simulink model "example"  (R2022a)
settings: Solver=VariableStepAuto  StartTime=0.0  StopTime=10.0  RelTol=1e-3
libraries: kif2 x289
settings Model: Creator=Felhasználó  LastModifiedBy=Felhasználó

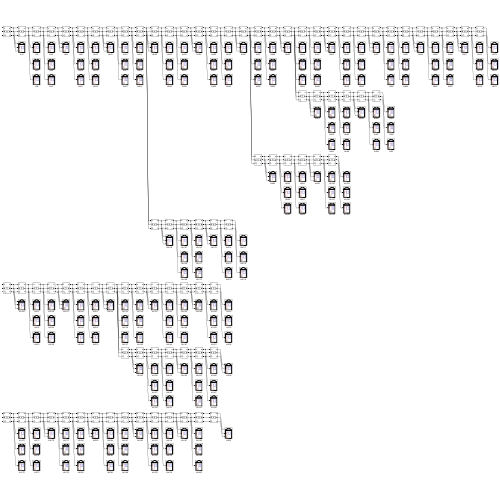
[thumbnail: Simulink's stored preview of the top-level diagram]
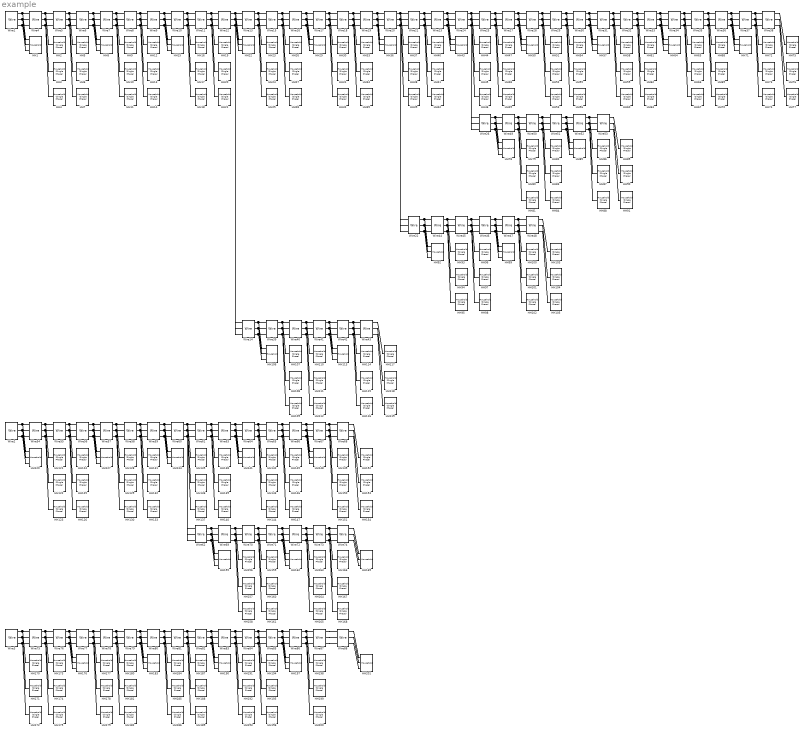
== system example ==
  HH1 : kif2/Household  Ctag=CONS7  Atag=Signal  Itag=Irrad  Ttag=T_Amb  Wtag=Wind  HHtag=PQ_HH1  HHtagv=global  PVtag=PQ_PV1  PVtagv=global  EStag=PQ_ES1  EStagv=global  HPtag=PQ_HP1  HPtagv=global
      link override ES: Cap=36500  SoCin=0.8  Pin=17300  Pout=-17300
      link override HP: P_HP=4800  C=5220  H=284
      link override PV: P_STCm=3100
      settings: SourceProductName=KIF2 Library
  HH10 : kif2/Household (Single Phase)  Ctag=CONS2  Atag=Signal  Itag=Irrad  Ttag=T_Amb  Wtag=Wind  HHtag=PQ_HH10  HHtagv=global  PVtag=PQ_PV10  PVtagv=global  EStag=PQ_ES10  EStagv=global  HPtag=PQ_HP10  HPtagv=global
      link override ES: Cap=13700  SoCin=0.3  Pin=7300  Pout=-7300
      link override HP: P_HP=3000  C=4950  H=141
      link override PV: P_STCm=1200
      settings: SourceProductName=KIF2 Library
  HH100 : kif2/Household (Single Phase)  Ctag=CONS1  Atag=Signal  Itag=Irrad  Ttag=T_Amb  Wtag=Wind  HHtag=PQ_HH100  HHtagv=global  PVtag=PQ_PV100  PVtagv=global  EStag=PQ_ES100  EStagv=global  HPtag=PQ_HP100  HPtagv=global
      link override ES: Cap=9100  SoCin=0.2  Pin=5300  Pout=-5300
      link override HP: P_HP=2400  C=2655  H=140
      link override PV: P_STCm=800
      settings: SourceProductName=KIF2 Library
  HH101 : kif2/Household (Single Phase)  Ctag=CONS2  Atag=Signal  Itag=Irrad  Ttag=T_Amb  Wtag=Wind  HHtag=PQ_HH101  HHtagv=global  PVtag=PQ_PV101  PVtagv=global  EStag=PQ_ES101  EStagv=global  HPtag=PQ_HP101  HPtagv=global
      link override ES: Cap=13700  SoCin=0.3  Pin=7300  Pout=-7300
      link override HP: P_HP=3000  C=4950  H=141
      link override PV: P_STCm=1200
      settings: SourceProductName=KIF2 Library
  HH102 : kif2/Household (Single Phase)  Ctag=CONS3  Atag=Signal  Itag=Irrad  Ttag=T_Amb  Wtag=Wind  HHtag=PQ_HH102  HHtagv=global  PVtag=PQ_PV102  PVtagv=global  EStag=PQ_ES102  EStagv=global  HPtag=PQ_HP102  HPtagv=global
      link override ES: Cap=18300  SoCin=0.4  Pin=9300  Pout=-9300
      link override HP: P_HP=2500  C=2520  H=146
      link override PV: P_STCm=1500
      settings: SourceProductName=KIF2 Library
  HH103 : kif2/Household (Single Phase)  Ctag=CONS4  Atag=Signal  Itag=Irrad  Ttag=T_Amb  Wtag=Wind  HHtag=PQ_HH103  HHtagv=global  PVtag=PQ_PV103  PVtagv=global  EStag=PQ_ES103  EStagv=global  HPtag=PQ_HP103  HPtagv=global
      link override ES: Cap=22800  Pin=11300  Pout=-11300
      link override HP: P_HP=3300  C=4635  H=176
      link override PV: P_STCm=1900
      settings: SourceProductName=KIF2 Library
  HH104 : kif2/Household (Single Phase)  Ctag=CONS5  Atag=Signal  Itag=Irrad  Ttag=T_Amb  Wtag=Wind  HHtag=PQ_HH104  HHtagv=global  PVtag=PQ_PV104  PVtagv=global  EStag=PQ_ES104  EStagv=global  HPtag=PQ_HP104  HPtagv=global
      link override ES: Cap=27400  SoCin=0.6  Pin=13300  Pout=-13300
      link override PV: P_STCm=2300
      settings: SourceProductName=KIF2 Library
  HH105 : kif2/Household (Single Phase)  Ctag=CONS6  Atag=Signal  Itag=Irrad  Ttag=T_Amb  Wtag=Wind  HHtag=PQ_HH105  HHtagv=global  PVtag=PQ_PV105  PVtagv=global  EStag=PQ_ES105  EStagv=global  HPtag=PQ_HP105  HPtagv=global
      link override ES: Cap=32000  SoCin=0.7  Pin=15300  Pout=-15300
      link override HP: P_HP=4200  C=4590  H=241
      settings: SourceProductName=KIF2 Library
  HH106 : kif2/Household  Ctag=CONS7  Atag=Signal  Itag=Irrad  Ttag=T_Amb  Wtag=Wind  HHtag=PQ_HH106  HHtagv=global  PVtag=PQ_PV106  PVtagv=global  EStag=PQ_ES106  EStagv=global  HPtag=PQ_HP106  HPtagv=global
      link override ES: Cap=36500  SoCin=0.8  Pin=17300  Pout=-17300
      link override HP: P_HP=4800  C=5220  H=284
      link override PV: P_STCm=3100
      settings: SourceProductName=KIF2 Library
  HH107 : kif2/Household (Single Phase)  Ctag=CONS1  Atag=Signal  Itag=Irrad  Ttag=T_Amb  Wtag=Wind  HHtag=PQ_HH107  HHtagv=global  PVtag=PQ_PV107  PVtagv=global  EStag=PQ_ES107  EStagv=global  HPtag=PQ_HP107  HPtagv=global
      link override ES: Cap=9100  SoCin=0.2  Pin=5300  Pout=-5300
      link override HP: P_HP=2400  C=2655  H=140
      link override PV: P_STCm=800
      settings: SourceProductName=KIF2 Library
  HH108 : kif2/Household (Single Phase)  Ctag=CONS2  Atag=Signal  Itag=Irrad  Ttag=T_Amb  Wtag=Wind  HHtag=PQ_HH108  HHtagv=global  PVtag=PQ_PV108  PVtagv=global  EStag=PQ_ES108  EStagv=global  HPtag=PQ_HP108  HPtagv=global
      link override ES: Cap=13700  SoCin=0.3  Pin=7300  Pout=-7300
      link override HP: P_HP=3000  C=4950  H=141
      link override PV: P_STCm=1200
      settings: SourceProductName=KIF2 Library
  HH109 : kif2/Household (Single Phase)  Ctag=CONS3  Atag=Signal  Itag=Irrad  Ttag=T_Amb  Wtag=Wind  HHtag=PQ_HH109  HHtagv=global  PVtag=PQ_PV109  PVtagv=global  EStag=PQ_ES109  EStagv=global  HPtag=PQ_HP109  HPtagv=global
      link override ES: Cap=18300  SoCin=0.4  Pin=9300  Pout=-9300
      link override HP: P_HP=2500  C=2520  H=146
      link override PV: P_STCm=1500
      settings: SourceProductName=KIF2 Library
  HH11 : kif2/Household (Single Phase)  Ctag=CONS3  Atag=Signal  Itag=Irrad  Ttag=T_Amb  Wtag=Wind  HHtag=PQ_HH11  HHtagv=global  PVtag=PQ_PV11  PVtagv=global  EStag=PQ_ES11  EStagv=global  HPtag=PQ_HP11  HPtagv=global
      link override ES: Cap=18300  SoCin=0.4  Pin=9300  Pout=-9300
      link override HP: P_HP=2500  C=2520  H=146
      link override PV: P_STCm=1500
      settings: SourceProductName=KIF2 Library
  HH110 : kif2/Household (Single Phase)  Ctag=CONS4  Atag=Signal  Itag=Irrad  Ttag=T_Amb  Wtag=Wind  HHtag=PQ_HH110  HHtagv=global  PVtag=PQ_PV110  PVtagv=global  EStag=PQ_ES110  EStagv=global  HPtag=PQ_HP110  HPtagv=global
      link override ES: Cap=22800  Pin=11300  Pout=-11300
      link override HP: P_HP=3300  C=4635  H=176
      link override PV: P_STCm=1900
      settings: SourceProductName=KIF2 Library
  HH111 : kif2/Household (Single Phase)  Ctag=CONS5  Atag=Signal  Itag=Irrad  Ttag=T_Amb  Wtag=Wind  HHtag=PQ_HH111  HHtagv=global  PVtag=PQ_PV111  PVtagv=global  EStag=PQ_ES111  EStagv=global  HPtag=PQ_HP111  HPtagv=global
      link override ES: Cap=27400  SoCin=0.6  Pin=13300  Pout=-13300
      link override PV: P_STCm=2300
      settings: SourceProductName=KIF2 Library
  HH112 : kif2/Household (Single Phase)  Ctag=CONS6  Atag=Signal  Itag=Irrad  Ttag=T_Amb  Wtag=Wind  HHtag=PQ_HH112  HHtagv=global  PVtag=PQ_PV112  PVtagv=global  EStag=PQ_ES112  EStagv=global  HPtag=PQ_HP112  HPtagv=global
      link override ES: Cap=32000  SoCin=0.7  Pin=15300  Pout=-15300
      link override HP: P_HP=4200  C=4590  H=241
      settings: SourceProductName=KIF2 Library
  HH113 : kif2/Household  Ctag=CONS7  Atag=Signal  Itag=Irrad  Ttag=T_Amb  Wtag=Wind  HHtag=PQ_HH113  HHtagv=global  PVtag=PQ_PV113  PVtagv=global  EStag=PQ_ES113  EStagv=global  HPtag=PQ_HP113  HPtagv=global
      link override ES: Cap=36500  SoCin=0.8  Pin=17300  Pout=-17300
      link override HP: P_HP=4800  C=5220  H=284
      link override PV: P_STCm=3100
      settings: SourceProductName=KIF2 Library
  HH114 : kif2/Household (Single Phase)  Ctag=CONS1  Atag=Signal  Itag=Irrad  Ttag=T_Amb  Wtag=Wind  HHtag=PQ_HH114  HHtagv=global  PVtag=PQ_PV114  PVtagv=global  EStag=PQ_ES114  EStagv=global  HPtag=PQ_HP114  HPtagv=global
      link override ES: Cap=9100  SoCin=0.2  Pin=5300  Pout=-5300
      link override HP: P_HP=2400  C=2655  H=140
      link override PV: P_STCm=800
      settings: SourceProductName=KIF2 Library
  HH115 : kif2/Household (Single Phase)  Ctag=CONS2  Atag=Signal  Itag=Irrad  Ttag=T_Amb  Wtag=Wind  HHtag=PQ_HH115  HHtagv=global  PVtag=PQ_PV115  PVtagv=global  EStag=PQ_ES115  EStagv=global  HPtag=PQ_HP115  HPtagv=global
      link override ES: Cap=13700  SoCin=0.3  Pin=7300  Pout=-7300
      link override HP: P_HP=3000  C=4950  H=141
      link override PV: P_STCm=1200
      settings: SourceProductName=KIF2 Library
  HH116 : kif2/Household (Single Phase)  Ctag=CONS3  Atag=Signal  Itag=Irrad  Ttag=T_Amb  Wtag=Wind  HHtag=PQ_HH116  HHtagv=global  PVtag=PQ_PV116  PVtagv=global  EStag=PQ_ES116  EStagv=global  HPtag=PQ_HP116  HPtagv=global
      link override ES: Cap=18300  SoCin=0.4  Pin=9300  Pout=-9300
      link override HP: P_HP=2500  C=2520  H=146
      link override PV: P_STCm=1500
      settings: SourceProductName=KIF2 Library
  HH117 : kif2/Household (Single Phase)  Ctag=CONS4  Atag=Signal  Itag=Irrad  Ttag=T_Amb  Wtag=Wind  HHtag=PQ_HH117  HHtagv=global  PVtag=PQ_PV117  PVtagv=global  EStag=PQ_ES117  EStagv=global  HPtag=PQ_HP117  HPtagv=global
      link override ES: Cap=22800  Pin=11300  Pout=-11300
      link override HP: P_HP=3300  C=4635  H=176
      link override PV: P_STCm=1900
      settings: SourceProductName=KIF2 Library
  HH118 : kif2/Household (Single Phase)  Ctag=CONS5  Atag=Signal  Itag=Irrad  Ttag=T_Amb  Wtag=Wind  HHtag=PQ_HH118  HHtagv=global  PVtag=PQ_PV118  PVtagv=global  EStag=PQ_ES118  EStagv=global  HPtag=PQ_HP118  HPtagv=global
      link override ES: Cap=27400  SoCin=0.6  Pin=13300  Pout=-13300
      link override PV: P_STCm=2300
      settings: SourceProductName=KIF2 Library
  HH119 : kif2/Household (Single Phase)  Ctag=CONS6  Atag=Signal  Itag=Irrad  Ttag=T_Amb  Wtag=Wind  HHtag=PQ_HH119  HHtagv=global  PVtag=PQ_PV119  PVtagv=global  EStag=PQ_ES119  EStagv=global  HPtag=PQ_HP119  HPtagv=global
      link override ES: Cap=32000  SoCin=0.7  Pin=15300  Pout=-15300
      link override HP: P_HP=4200  C=4590  H=241
      settings: SourceProductName=KIF2 Library
  HH12 : kif2/Household (Single Phase)  Ctag=CONS4  Atag=Signal  Itag=Irrad  Ttag=T_Amb  Wtag=Wind  HHtag=PQ_HH12  HHtagv=global  PVtag=PQ_PV12  PVtagv=global  EStag=PQ_ES12  EStagv=global  HPtag=PQ_HP12  HPtagv=global
      link override ES: Cap=22800  Pin=11300  Pout=-11300
      link override HP: P_HP=3300  C=4635  H=176
      link override PV: P_STCm=1900
      settings: SourceProductName=KIF2 Library
  HH120 : kif2/Household  Ctag=CONS7  Atag=Signal  Itag=Irrad  Ttag=T_Amb  Wtag=Wind  HHtag=PQ_HH120  HHtagv=global  PVtag=PQ_PV120  PVtagv=global  EStag=PQ_ES120  EStagv=global  HPtag=PQ_HP120  HPtagv=global
      link override ES: Cap=36500  SoCin=0.8  Pin=17300  Pout=-17300
      link override HP: P_HP=4800  C=5220  H=284
      link override PV: P_STCm=3100
      settings: SourceProductName=KIF2 Library
  HH121 : kif2/Household (Single Phase)  Ctag=CONS1  Atag=Signal  Itag=Irrad  Ttag=T_Amb  Wtag=Wind  HHtag=PQ_HH121  HHtagv=global  PVtag=PQ_PV121  PVtagv=global  EStag=PQ_ES121  EStagv=global  HPtag=PQ_HP121  HPtagv=global
      link override ES: Cap=9100  SoCin=0.2  Pin=5300  Pout=-5300
      link override HP: P_HP=2400  C=2655  H=140
      link override PV: P_STCm=800
      settings: SourceProductName=KIF2 Library
  HH122 : kif2/Household (Single Phase)  Ctag=CONS2  Atag=Signal  Itag=Irrad  Ttag=T_Amb  Wtag=Wind  HHtag=PQ_HH122  HHtagv=global  PVtag=PQ_PV122  PVtagv=global  EStag=PQ_ES122  EStagv=global  HPtag=PQ_HP122  HPtagv=global
      link override ES: Cap=13700  SoCin=0.3  Pin=7300  Pout=-7300
      link override HP: P_HP=3000  C=4950  H=141
      link override PV: P_STCm=1200
      settings: SourceProductName=KIF2 Library
  HH123 : kif2/Household (Single Phase)  Ctag=CONS3  Atag=Signal  Itag=Irrad  Ttag=T_Amb  Wtag=Wind  HHtag=PQ_HH123  HHtagv=global  PVtag=PQ_PV123  PVtagv=global  EStag=PQ_ES123  EStagv=global  HPtag=PQ_HP123  HPtagv=global
      link override ES: Cap=18300  SoCin=0.4  Pin=9300  Pout=-9300
      link override HP: P_HP=2500  C=2520  H=146
      link override PV: P_STCm=1500
      settings: SourceProductName=KIF2 Library
  HH124 : kif2/Household (Single Phase)  Ctag=CONS4  Atag=Signal  Itag=Irrad  Ttag=T_Amb  Wtag=Wind  HHtag=PQ_HH124  HHtagv=global  PVtag=PQ_PV124  PVtagv=global  EStag=PQ_ES124  EStagv=global  HPtag=PQ_HP124  HPtagv=global
      link override ES: Cap=22800  Pin=11300  Pout=-11300
      link override HP: P_HP=3300  C=4635  H=176
      link override PV: P_STCm=1900
      settings: SourceProductName=KIF2 Library
  HH125 : kif2/Household (Single Phase)  Ctag=CONS5  Atag=Signal  Itag=Irrad  Ttag=T_Amb  Wtag=Wind  HHtag=PQ_HH125  HHtagv=global  PVtag=PQ_PV125  PVtagv=global  EStag=PQ_ES125  EStagv=global  HPtag=PQ_HP125  HPtagv=global
      link override ES: Cap=27400  SoCin=0.6  Pin=13300  Pout=-13300
      link override PV: P_STCm=2300
      settings: SourceProductName=KIF2 Library
  HH126 : kif2/Household (Single Phase)  Ctag=CONS6  Atag=Signal  Itag=Irrad  Ttag=T_Amb  Wtag=Wind  HHtag=PQ_HH126  HHtagv=global  PVtag=PQ_PV126  PVtagv=global  EStag=PQ_ES126  EStagv=global  HPtag=PQ_HP126  HPtagv=global
      link override ES: Cap=32000  SoCin=0.7  Pin=15300  Pout=-15300
      link override HP: P_HP=4200  C=4590  H=241
      settings: SourceProductName=KIF2 Library
  HH127 : kif2/Household  Ctag=CONS7  Atag=Signal  Itag=Irrad  Ttag=T_Amb  Wtag=Wind  HHtag=PQ_HH127  HHtagv=global  PVtag=PQ_PV127  PVtagv=global  EStag=PQ_ES127  EStagv=global  HPtag=PQ_HP127  HPtagv=global
      link override ES: Cap=36500  SoCin=0.8  Pin=17300  Pout=-17300
      link override HP: P_HP=4800  C=5220  H=284
      link override PV: P_STCm=3100
      settings: SourceProductName=KIF2 Library
  HH128 : kif2/Household (Single Phase)  Ctag=CONS1  Atag=Signal  Itag=Irrad  Ttag=T_Amb  Wtag=Wind  HHtag=PQ_HH128  HHtagv=global  PVtag=PQ_PV128  PVtagv=global  EStag=PQ_ES128  EStagv=global  HPtag=PQ_HP128  HPtagv=global
      link override ES: Cap=9100  SoCin=0.2  Pin=5300  Pout=-5300
      link override HP: P_HP=2400  C=2655  H=140
      link override PV: P_STCm=800
      settings: SourceProductName=KIF2 Library
  HH129 : kif2/Household (Single Phase)  Ctag=CONS2  Atag=Signal  Itag=Irrad  Ttag=T_Amb  Wtag=Wind  HHtag=PQ_HH129  HHtagv=global  PVtag=PQ_PV129  PVtagv=global  EStag=PQ_ES129  EStagv=global  HPtag=PQ_HP129  HPtagv=global
      link override ES: Cap=13700  SoCin=0.3  Pin=7300  Pout=-7300
      link override HP: P_HP=3000  C=4950  H=141
      link override PV: P_STCm=1200
      settings: SourceProductName=KIF2 Library
  HH13 : kif2/Household (Single Phase)  Ctag=CONS5  Atag=Signal  Itag=Irrad  Ttag=T_Amb  Wtag=Wind  HHtag=PQ_HH13  HHtagv=global  PVtag=PQ_PV13  PVtagv=global  EStag=PQ_ES13  EStagv=global  HPtag=PQ_HP13  HPtagv=global
      link override ES: Cap=27400  SoCin=0.6  Pin=13300  Pout=-13300
      link override PV: P_STCm=2300
      settings: SourceProductName=KIF2 Library
  HH130 : kif2/Household (Single Phase)  Ctag=CONS3  Atag=Signal  Itag=Irrad  Ttag=T_Amb  Wtag=Wind  HHtag=PQ_HH130  HHtagv=global  PVtag=PQ_PV130  PVtagv=global  EStag=PQ_ES130  EStagv=global  HPtag=PQ_HP130  HPtagv=global
      link override ES: Cap=18300  SoCin=0.4  Pin=9300  Pout=-9300
      link override HP: P_HP=2500  C=2520  H=146
      link override PV: P_STCm=1500
      settings: SourceProductName=KIF2 Library
  HH131 : kif2/Household (Single Phase)  Ctag=CONS4  Atag=Signal  Itag=Irrad  Ttag=T_Amb  Wtag=Wind  HHtag=PQ_HH131  HHtagv=global  PVtag=PQ_PV131  PVtagv=global  EStag=PQ_ES131  EStagv=global  HPtag=PQ_HP131  HPtagv=global
      link override ES: Cap=22800  Pin=11300  Pout=-11300
      link override HP: P_HP=3300  C=4635  H=176
      link override PV: P_STCm=1900
      settings: SourceProductName=KIF2 Library
  HH132 : kif2/Household (Single Phase)  Ctag=CONS5  Atag=Signal  Itag=Irrad  Ttag=T_Amb  Wtag=Wind  HHtag=PQ_HH132  HHtagv=global  PVtag=PQ_PV132  PVtagv=global  EStag=PQ_ES132  EStagv=global  HPtag=PQ_HP132  HPtagv=global
      link override ES: Cap=27400  SoCin=0.6  Pin=13300  Pout=-13300
      link override PV: P_STCm=2300
      settings: SourceProductName=KIF2 Library
  HH133 : kif2/Household (Single Phase)  Ctag=CONS6  Atag=Signal  Itag=Irrad  Ttag=T_Amb  Wtag=Wind  HHtag=PQ_HH133  HHtagv=global  PVtag=PQ_PV133  PVtagv=global  EStag=PQ_ES133  EStagv=global  HPtag=PQ_HP133  HPtagv=global
      link override ES: Cap=32000  SoCin=0.7  Pin=15300  Pout=-15300
      link override HP: P_HP=4200  C=4590  H=241
      settings: SourceProductName=KIF2 Library
  HH134 : kif2/Household  Ctag=CONS7  Atag=Signal  Itag=Irrad  Ttag=T_Amb  Wtag=Wind  HHtag=PQ_HH134  HHtagv=global  PVtag=PQ_PV134  PVtagv=global  EStag=PQ_ES134  EStagv=global  HPtag=PQ_HP134  HPtagv=global
      link override ES: Cap=36500  SoCin=0.8  Pin=17300  Pout=-17300
      link override HP: P_HP=4800  C=5220  H=284
      link override PV: P_STCm=3100
      settings: SourceProductName=KIF2 Library
  HH135 : kif2/Household (Single Phase)  Ctag=CONS1  Atag=Signal  Itag=Irrad  Ttag=T_Amb  Wtag=Wind  HHtag=PQ_HH135  HHtagv=global  PVtag=PQ_PV135  PVtagv=global  EStag=PQ_ES135  EStagv=global  HPtag=PQ_HP135  HPtagv=global
      link override ES: Cap=9100  SoCin=0.2  Pin=5300  Pout=-5300
      link override HP: P_HP=2400  C=2655  H=140
      link override PV: P_STCm=800
      settings: SourceProductName=KIF2 Library
  HH136 : kif2/Household (Single Phase)  Ctag=CONS2  Atag=Signal  Itag=Irrad  Ttag=T_Amb  Wtag=Wind  HHtag=PQ_HH136  HHtagv=global  PVtag=PQ_PV136  PVtagv=global  EStag=PQ_ES136  EStagv=global  HPtag=PQ_HP136  HPtagv=global
      link override ES: Cap=13700  SoCin=0.3  Pin=7300  Pout=-7300
      link override HP: P_HP=3000  C=4950  H=141
      link override PV: P_STCm=1200
      settings: SourceProductName=KIF2 Library
  HH137 : kif2/Household (Single Phase)  Ctag=CONS3  Atag=Signal  Itag=Irrad  Ttag=T_Amb  Wtag=Wind  HHtag=PQ_HH137  HHtagv=global  PVtag=PQ_PV137  PVtagv=global  EStag=PQ_ES137  EStagv=global  HPtag=PQ_HP137  HPtagv=global
      link override ES: Cap=18300  SoCin=0.4  Pin=9300  Pout=-9300
      link override HP: P_HP=2500  C=2520  H=146
      link override PV: P_STCm=1500
      settings: SourceProductName=KIF2 Library
  HH138 : kif2/Household (Single Phase)  Ctag=CONS4  Atag=Signal  Itag=Irrad  Ttag=T_Amb  Wtag=Wind  HHtag=PQ_HH138  HHtagv=global  PVtag=PQ_PV138  PVtagv=global  EStag=PQ_ES138  EStagv=global  HPtag=PQ_HP138  HPtagv=global
      link override ES: Cap=22800  Pin=11300  Pout=-11300
      link override HP: P_HP=3300  C=4635  H=176
      link override PV: P_STCm=1900
      settings: SourceProductName=KIF2 Library
  HH139 : kif2/Household (Single Phase)  Ctag=CONS5  Atag=Signal  Itag=Irrad  Ttag=T_Amb  Wtag=Wind  HHtag=PQ_HH139  HHtagv=global  PVtag=PQ_PV139  PVtagv=global  EStag=PQ_ES139  EStagv=global  HPtag=PQ_HP139  HPtagv=global
      link override ES: Cap=27400  SoCin=0.6  Pin=13300  Pout=-13300
      link override PV: P_STCm=2300
      settings: SourceProductName=KIF2 Library
  HH14 : kif2/Household (Single Phase)  Ctag=CONS6  Atag=Signal  Itag=Irrad  Ttag=T_Amb  Wtag=Wind  HHtag=PQ_HH14  HHtagv=global  PVtag=PQ_PV14  PVtagv=global  EStag=PQ_ES14  EStagv=global  HPtag=PQ_HP14  HPtagv=global
      link override ES: Cap=32000  SoCin=0.7  Pin=15300  Pout=-15300
      link override HP: P_HP=4200  C=4590  H=241
      settings: SourceProductName=KIF2 Library
  HH140 : kif2/Household (Single Phase)  Ctag=CONS6  Atag=Signal  Itag=Irrad  Ttag=T_Amb  Wtag=Wind  HHtag=PQ_HH140  HHtagv=global  PVtag=PQ_PV140  PVtagv=global  EStag=PQ_ES140  EStagv=global  HPtag=PQ_HP140  HPtagv=global
      link override ES: Cap=32000  SoCin=0.7  Pin=15300  Pout=-15300
      link override HP: P_HP=4200  C=4590  H=241
      settings: SourceProductName=KIF2 Library
  HH141 : kif2/Household  Ctag=CONS7  Atag=Signal  Itag=Irrad  Ttag=T_Amb  Wtag=Wind  HHtag=PQ_HH141  HHtagv=global  PVtag=PQ_PV141  PVtagv=global  EStag=PQ_ES141  EStagv=global  HPtag=PQ_HP141  HPtagv=global
      link override ES: Cap=36500  SoCin=0.8  Pin=17300  Pout=-17300
      link override HP: P_HP=4800  C=5220  H=284
      link override PV: P_STCm=3100
      settings: SourceProductName=KIF2 Library
  HH142 : kif2/Household (Single Phase)  Ctag=CONS1  Atag=Signal  Itag=Irrad  Ttag=T_Amb  Wtag=Wind  HHtag=PQ_HH142  HHtagv=global  PVtag=PQ_PV142  PVtagv=global  EStag=PQ_ES142  EStagv=global  HPtag=PQ_HP142  HPtagv=global
      link override ES: Cap=9100  SoCin=0.2  Pin=5300  Pout=-5300
      link override HP: P_HP=2400  C=2655  H=140
      link override PV: P_STCm=800
      settings: SourceProductName=KIF2 Library
  HH143 : kif2/Household (Single Phase)  Ctag=CONS2  Atag=Signal  Itag=Irrad  Ttag=T_Amb  Wtag=Wind  HHtag=PQ_HH143  HHtagv=global  PVtag=PQ_PV143  PVtagv=global  EStag=PQ_ES143  EStagv=global  HPtag=PQ_HP143  HPtagv=global
      link override ES: Cap=13700  SoCin=0.3  Pin=7300  Pout=-7300
      link override HP: P_HP=3000  C=4950  H=141
      link override PV: P_STCm=1200
      settings: SourceProductName=KIF2 Library
  HH144 : kif2/Household (Single Phase)  Ctag=CONS3  Atag=Signal  Itag=Irrad  Ttag=T_Amb  Wtag=Wind  HHtag=PQ_HH144  HHtagv=global  PVtag=PQ_PV144  PVtagv=global  EStag=PQ_ES144  EStagv=global  HPtag=PQ_HP144  HPtagv=global
      link override ES: Cap=18300  SoCin=0.4  Pin=9300  Pout=-9300
      link override HP: P_HP=2500  C=2520  H=146
      link override PV: P_STCm=1500
      settings: SourceProductName=KIF2 Library
  HH145 : kif2/Household (Single Phase)  Ctag=CONS4  Atag=Signal  Itag=Irrad  Ttag=T_Amb  Wtag=Wind  HHtag=PQ_HH145  HHtagv=global  PVtag=PQ_PV145  PVtagv=global  EStag=PQ_ES145  EStagv=global  HPtag=PQ_HP145  HPtagv=global
      link override ES: Cap=22800  Pin=11300  Pout=-11300
      link override HP: P_HP=3300  C=4635  H=176
      link override PV: P_STCm=1900
      settings: SourceProductName=KIF2 Library
  HH146 : kif2/Household (Single Phase)  Ctag=CONS5  Atag=Signal  Itag=Irrad  Ttag=T_Amb  Wtag=Wind  HHtag=PQ_HH146  HHtagv=global  PVtag=PQ_PV146  PVtagv=global  EStag=PQ_ES146  EStagv=global  HPtag=PQ_HP146  HPtagv=global
      link override ES: Cap=27400  SoCin=0.6  Pin=13300  Pout=-13300
      link override PV: P_STCm=2300
      settings: SourceProductName=KIF2 Library
  HH147 : kif2/Household (Single Phase)  Ctag=CONS6  Atag=Signal  Itag=Irrad  Ttag=T_Amb  Wtag=Wind  HHtag=PQ_HH147  HHtagv=global  PVtag=PQ_PV147  PVtagv=global  EStag=PQ_ES147  EStagv=global  HPtag=PQ_HP147  HPtagv=global
      link override ES: Cap=32000  SoCin=0.7  Pin=15300  Pout=-15300
      link override HP: P_HP=4200  C=4590  H=241
      settings: SourceProductName=KIF2 Library
  HH148 : kif2/Household  Ctag=CONS7  Atag=Signal  Itag=Irrad  Ttag=T_Amb  Wtag=Wind  HHtag=PQ_HH148  HHtagv=global  PVtag=PQ_PV148  PVtagv=global  EStag=PQ_ES148  EStagv=global  HPtag=PQ_HP148  HPtagv=global
      link override ES: Cap=36500  SoCin=0.8  Pin=17300  Pout=-17300
      link override HP: P_HP=4800  C=5220  H=284
      link override PV: P_STCm=3100
      settings: SourceProductName=KIF2 Library
  HH149 : kif2/Household (Single Phase)  Ctag=CONS1  Atag=Signal  Itag=Irrad  Ttag=T_Amb  Wtag=Wind  HHtag=PQ_HH149  HHtagv=global  PVtag=PQ_PV149  PVtagv=global  EStag=PQ_ES149  EStagv=global  HPtag=PQ_HP149  HPtagv=global
      link override ES: Cap=9100  SoCin=0.2  Pin=5300  Pout=-5300
      link override HP: P_HP=2400  C=2655  H=140
      link override PV: P_STCm=800
      settings: SourceProductName=KIF2 Library
  HH15 : kif2/Household  Ctag=CONS7  Atag=Signal  Itag=Irrad  Ttag=T_Amb  Wtag=Wind  HHtag=PQ_HH15  HHtagv=global  PVtag=PQ_PV15  PVtagv=global  EStag=PQ_ES15  EStagv=global  HPtag=PQ_HP15  HPtagv=global
      link override ES: Cap=36500  SoCin=0.8  Pin=17300  Pout=-17300
      link override HP: P_HP=4800  C=5220  H=284
      link override PV: P_STCm=3100
      settings: SourceProductName=KIF2 Library
  HH150 : kif2/Household (Single Phase)  Ctag=CONS2  Atag=Signal  Itag=Irrad  Ttag=T_Amb  Wtag=Wind  HHtag=PQ_HH150  HHtagv=global  PVtag=PQ_PV150  PVtagv=global  EStag=PQ_ES150  EStagv=global  HPtag=PQ_HP150  HPtagv=global
      link override ES: Cap=13700  SoCin=0.3  Pin=7300  Pout=-7300
      link override HP: P_HP=3000  C=4950  H=141
      link override PV: P_STCm=1200
      settings: SourceProductName=KIF2 Library
  HH151 : kif2/Household (Single Phase)  Ctag=CONS3  Atag=Signal  Itag=Irrad  Ttag=T_Amb  Wtag=Wind  HHtag=PQ_HH151  HHtagv=global  PVtag=PQ_PV151  PVtagv=global  EStag=PQ_ES151  EStagv=global  HPtag=PQ_HP151  HPtagv=global
      link override ES: Cap=18300  SoCin=0.4  Pin=9300  Pout=-9300
      link override HP: P_HP=2500  C=2520  H=146
      link override PV: P_STCm=1500
      settings: SourceProductName=KIF2 Library
  HH152 : kif2/Household (Single Phase)  Ctag=CONS4  Atag=Signal  Itag=Irrad  Ttag=T_Amb  Wtag=Wind  HHtag=PQ_HH152  HHtagv=global  PVtag=PQ_PV152  PVtagv=global  EStag=PQ_ES152  EStagv=global  HPtag=PQ_HP152  HPtagv=global
      link override ES: Cap=22800  Pin=11300  Pout=-11300
      link override HP: P_HP=3300  C=4635  H=176
      link override PV: P_STCm=1900
      settings: SourceProductName=KIF2 Library
  HH153 : kif2/Household (Single Phase)  Ctag=CONS5  Atag=Signal  Itag=Irrad  Ttag=T_Amb  Wtag=Wind  HHtag=PQ_HH153  HHtagv=global  PVtag=PQ_PV153  PVtagv=global  EStag=PQ_ES153  EStagv=global  HPtag=PQ_HP153  HPtagv=global
      link override ES: Cap=27400  SoCin=0.6  Pin=13300  Pout=-13300
      link override PV: P_STCm=2300
      settings: SourceProductName=KIF2 Library
  HH154 : kif2/Household (Single Phase)  Ctag=CONS6  Atag=Signal  Itag=Irrad  Ttag=T_Amb  Wtag=Wind  HHtag=PQ_HH154  HHtagv=global  PVtag=PQ_PV154  PVtagv=global  EStag=PQ_ES154  EStagv=global  HPtag=PQ_HP154  HPtagv=global
      link override ES: Cap=32000  SoCin=0.7  Pin=15300  Pout=-15300
      link override HP: P_HP=4200  C=4590  H=241
      settings: SourceProductName=KIF2 Library
  HH155 : kif2/Household  Ctag=CONS7  Atag=Signal  Itag=Irrad  Ttag=T_Amb  Wtag=Wind  HHtag=PQ_HH155  HHtagv=global  PVtag=PQ_PV155  PVtagv=global  EStag=PQ_ES155  EStagv=global  HPtag=PQ_HP155  HPtagv=global
      link override ES: Cap=36500  SoCin=0.8  Pin=17300  Pout=-17300
      link override HP: P_HP=4800  C=5220  H=284
      link override PV: P_STCm=3100
      settings: SourceProductName=KIF2 Library
  HH156 : kif2/Household (Single Phase)  Ctag=CONS1  Atag=Signal  Itag=Irrad  Ttag=T_Amb  Wtag=Wind  HHtag=PQ_HH156  HHtagv=global  PVtag=PQ_PV156  PVtagv=global  EStag=PQ_ES156  EStagv=global  HPtag=PQ_HP156  HPtagv=global
      link override ES: Cap=9100  SoCin=0.2  Pin=5300  Pout=-5300
      link override HP: P_HP=2400  C=2655  H=140
      link override PV: P_STCm=800
      settings: SourceProductName=KIF2 Library
  HH157 : kif2/Household (Single Phase)  Ctag=CONS2  Atag=Signal  Itag=Irrad  Ttag=T_Amb  Wtag=Wind  HHtag=PQ_HH157  HHtagv=global  PVtag=PQ_PV157  PVtagv=global  EStag=PQ_ES157  EStagv=global  HPtag=PQ_HP157  HPtagv=global
      link override ES: Cap=13700  SoCin=0.3  Pin=7300  Pout=-7300
      link override HP: P_HP=3000  C=4950  H=141
      link override PV: P_STCm=1200
      settings: SourceProductName=KIF2 Library
  HH158 : kif2/Household (Single Phase)  Ctag=CONS3  Atag=Signal  Itag=Irrad  Ttag=T_Amb  Wtag=Wind  HHtag=PQ_HH158  HHtagv=global  PVtag=PQ_PV158  PVtagv=global  EStag=PQ_ES158  EStagv=global  HPtag=PQ_HP158  HPtagv=global
      link override ES: Cap=18300  SoCin=0.4  Pin=9300  Pout=-9300
      link override HP: P_HP=2500  C=2520  H=146
      link override PV: P_STCm=1500
      settings: SourceProductName=KIF2 Library
  HH159 : kif2/Household (Single Phase)  Ctag=CONS4  Atag=Signal  Itag=Irrad  Ttag=T_Amb  Wtag=Wind  HHtag=PQ_HH159  HHtagv=global  PVtag=PQ_PV159  PVtagv=global  EStag=PQ_ES159  EStagv=global  HPtag=PQ_HP159  HPtagv=global
      link override ES: Cap=22800  Pin=11300  Pout=-11300
      link override HP: P_HP=3300  C=4635  H=176
      link override PV: P_STCm=1900
      settings: SourceProductName=KIF2 Library
  HH16 : kif2/Household (Single Phase)  Ctag=CONS1  Atag=Signal  Itag=Irrad  Ttag=T_Amb  Wtag=Wind  HHtag=PQ_HH16  HHtagv=global  PVtag=PQ_PV16  PVtagv=global  EStag=PQ_ES16  EStagv=global  HPtag=PQ_HP16  HPtagv=global
      link override ES: Cap=9100  SoCin=0.2  Pin=5300  Pout=-5300
      link override HP: P_HP=2400  C=2655  H=140
      link override PV: P_STCm=800
      settings: SourceProductName=KIF2 Library
  HH160 : kif2/Household (Single Phase)  Ctag=CONS5  Atag=Signal  Itag=Irrad  Ttag=T_Amb  Wtag=Wind  HHtag=PQ_HH160  HHtagv=global  PVtag=PQ_PV160  PVtagv=global  EStag=PQ_ES160  EStagv=global  HPtag=PQ_HP160  HPtagv=global
      link override ES: Cap=27400  SoCin=0.6  Pin=13300  Pout=-13300
      link override PV: P_STCm=2300
      settings: SourceProductName=KIF2 Library
  HH161 : kif2/Household (Single Phase)  Ctag=CONS6  Atag=Signal  Itag=Irrad  Ttag=T_Amb  Wtag=Wind  HHtag=PQ_HH161  HHtagv=global  PVtag=PQ_PV161  PVtagv=global  EStag=PQ_ES161  EStagv=global  HPtag=PQ_HP161  HPtagv=global
      link override ES: Cap=32000  SoCin=0.7  Pin=15300  Pout=-15300
      link override HP: P_HP=4200  C=4590  H=241
      settings: SourceProductName=KIF2 Library
  HH162 : kif2/Household  Ctag=CONS7  Atag=Signal  Itag=Irrad  Ttag=T_Amb  Wtag=Wind  HHtag=PQ_HH162  HHtagv=global  PVtag=PQ_PV162  PVtagv=global  EStag=PQ_ES162  EStagv=global  HPtag=PQ_HP162  HPtagv=global
      link override ES: Cap=36500  SoCin=0.8  Pin=17300  Pout=-17300
      link override HP: P_HP=4800  C=5220  H=284
      link override PV: P_STCm=3100
      settings: SourceProductName=KIF2 Library
  HH163 : kif2/Household (Single Phase)  Ctag=CONS1  Atag=Signal  Itag=Irrad  Ttag=T_Amb  Wtag=Wind  HHtag=PQ_HH163  HHtagv=global  PVtag=PQ_PV163  PVtagv=global  EStag=PQ_ES163  EStagv=global  HPtag=PQ_HP163  HPtagv=global
      link override ES: Cap=9100  SoCin=0.2  Pin=5300  Pout=-5300
      link override HP: P_HP=2400  C=2655  H=140
      link override PV: P_STCm=800
      settings: SourceProductName=KIF2 Library
  HH164 : kif2/Household (Single Phase)  Ctag=CONS2  Atag=Signal  Itag=Irrad  Ttag=T_Amb  Wtag=Wind  HHtag=PQ_HH164  HHtagv=global  PVtag=PQ_PV164  PVtagv=global  EStag=PQ_ES164  EStagv=global  HPtag=PQ_HP164  HPtagv=global
      link override ES: Cap=13700  SoCin=0.3  Pin=7300  Pout=-7300
      link override HP: P_HP=3000  C=4950  H=141
      link override PV: P_STCm=1200
      settings: SourceProductName=KIF2 Library
  HH165 : kif2/Household (Single Phase)  Ctag=CONS3  Atag=Signal  Itag=Irrad  Ttag=T_Amb  Wtag=Wind  HHtag=PQ_HH165  HHtagv=global  PVtag=PQ_PV165  PVtagv=global  EStag=PQ_ES165  EStagv=global  HPtag=PQ_HP165  HPtagv=global
      link override ES: Cap=18300  SoCin=0.4  Pin=9300  Pout=-9300
      link override HP: P_HP=2500  C=2520  H=146
      link override PV: P_STCm=1500
      settings: SourceProductName=KIF2 Library
  HH166 : kif2/Household (Single Phase)  Ctag=CONS4  Atag=Signal  Itag=Irrad  Ttag=T_Amb  Wtag=Wind  HHtag=PQ_HH166  HHtagv=global  PVtag=PQ_PV166  PVtagv=global  EStag=PQ_ES166  EStagv=global  HPtag=PQ_HP166  HPtagv=global
      link override ES: Cap=22800  Pin=11300  Pout=-11300
      link override HP: P_HP=3300  C=4635  H=176
      link override PV: P_STCm=1900
      settings: SourceProductName=KIF2 Library
  HH167 : kif2/Household (Single Phase)  Ctag=CONS5  Atag=Signal  Itag=Irrad  Ttag=T_Amb  Wtag=Wind  HHtag=PQ_HH167  HHtagv=global  PVtag=PQ_PV167  PVtagv=global  EStag=PQ_ES167  EStagv=global  HPtag=PQ_HP167  HPtagv=global
      link override ES: Cap=27400  SoCin=0.6  Pin=13300  Pout=-13300
      link override PV: P_STCm=2300
      settings: SourceProductName=KIF2 Library
  HH168 : kif2/Household (Single Phase)  Ctag=CONS6  Atag=Signal  Itag=Irrad  Ttag=T_Amb  Wtag=Wind  HHtag=PQ_HH168  HHtagv=global  PVtag=PQ_PV168  PVtagv=global  EStag=PQ_ES168  EStagv=global  HPtag=PQ_HP168  HPtagv=global
      link override ES: Cap=32000  SoCin=0.7  Pin=15300  Pout=-15300
      link override HP: P_HP=4200  C=4590  H=241
      settings: SourceProductName=KIF2 Library
  HH169 : kif2/Household  Ctag=CONS7  Atag=Signal  Itag=Irrad  Ttag=T_Amb  Wtag=Wind  HHtag=PQ_HH169  HHtagv=global  PVtag=PQ_PV169  PVtagv=global  EStag=PQ_ES169  EStagv=global  HPtag=PQ_HP169  HPtagv=global
      link override ES: Cap=36500  SoCin=0.8  Pin=17300  Pout=-17300
      link override HP: P_HP=4800  C=5220  H=284
      link override PV: P_STCm=3100
      settings: SourceProductName=KIF2 Library
  HH17 : kif2/Household (Single Phase)  Ctag=CONS2  Atag=Signal  Itag=Irrad  Ttag=T_Amb  Wtag=Wind  HHtag=PQ_HH17  HHtagv=global  PVtag=PQ_PV17  PVtagv=global  EStag=PQ_ES17  EStagv=global  HPtag=PQ_HP17  HPtagv=global
      link override ES: Cap=13700  SoCin=0.3  Pin=7300  Pout=-7300
      link override HP: P_HP=3000  C=4950  H=141
      link override PV: P_STCm=1200
      settings: SourceProductName=KIF2 Library
  HH170 : kif2/Household (Single Phase)  Ctag=CONS1  Atag=Signal  Itag=Irrad  Ttag=T_Amb  Wtag=Wind  HHtag=PQ_HH170  HHtagv=global  PVtag=PQ_PV170  PVtagv=global  EStag=PQ_ES170  EStagv=global  HPtag=PQ_HP170  HPtagv=global
      link override ES: Cap=9100  SoCin=0.2  Pin=5300  Pout=-5300
      link override HP: P_HP=2400  C=2655  H=140
      link override PV: P_STCm=800
      settings: SourceProductName=KIF2 Library
  HH171 : kif2/Household (Single Phase)  Ctag=CONS2  Atag=Signal  Itag=Irrad  Ttag=T_Amb  Wtag=Wind  HHtag=PQ_HH171  HHtagv=global  PVtag=PQ_PV171  PVtagv=global  EStag=PQ_ES171  EStagv=global  HPtag=PQ_HP171  HPtagv=global
      link override ES: Cap=13700  SoCin=0.3  Pin=7300  Pout=-7300
      link override HP: P_HP=3000  C=4950  H=141
      link override PV: P_STCm=1200
      settings: SourceProductName=KIF2 Library
  HH172 : kif2/Household (Single Phase)  Ctag=CONS3  Atag=Signal  Itag=Irrad  Ttag=T_Amb  Wtag=Wind  HHtag=PQ_HH172  HHtagv=global  PVtag=PQ_PV172  PVtagv=global  EStag=PQ_ES172  EStagv=global  HPtag=PQ_HP172  HPtagv=global
      link override ES: Cap=18300  SoCin=0.4  Pin=9300  Pout=-9300
      link override HP: P_HP=2500  C=2520  H=146
      link override PV: P_STCm=1500
      settings: SourceProductName=KIF2 Library
  HH173 : kif2/Household (Single Phase)  Ctag=CONS4  Atag=Signal  Itag=Irrad  Ttag=T_Amb  Wtag=Wind  HHtag=PQ_HH173  HHtagv=global  PVtag=PQ_PV173  PVtagv=global  EStag=PQ_ES173  EStagv=global  HPtag=PQ_HP173  HPtagv=global
      link override ES: Cap=22800  Pin=11300  Pout=-11300
      link override HP: P_HP=3300  C=4635  H=176
      link override PV: P_STCm=1900
      settings: SourceProductName=KIF2 Library
  HH174 : kif2/Household (Single Phase)  Ctag=CONS5  Atag=Signal  Itag=Irrad  Ttag=T_Amb  Wtag=Wind  HHtag=PQ_HH174  HHtagv=global  PVtag=PQ_PV174  PVtagv=global  EStag=PQ_ES174  EStagv=global  HPtag=PQ_HP174  HPtagv=global
      link override ES: Cap=27400  SoCin=0.6  Pin=13300  Pout=-13300
      link override PV: P_STCm=2300
      settings: SourceProductName=KIF2 Library
  HH175 : kif2/Household (Single Phase)  Ctag=CONS6  Atag=Signal  Itag=Irrad  Ttag=T_Amb  Wtag=Wind  HHtag=PQ_HH175  HHtagv=global  PVtag=PQ_PV175  PVtagv=global  EStag=PQ_ES175  EStagv=global  HPtag=PQ_HP175  HPtagv=global
      link override ES: Cap=32000  SoCin=0.7  Pin=15300  Pout=-15300
      link override HP: P_HP=4200  C=4590  H=241
      settings: SourceProductName=KIF2 Library
  HH176 : kif2/Household  Ctag=CONS7  Atag=Signal  Itag=Irrad  Ttag=T_Amb  Wtag=Wind  HHtag=PQ_HH176  HHtagv=global  PVtag=PQ_PV176  PVtagv=global  EStag=PQ_ES176  EStagv=global  HPtag=PQ_HP176  HPtagv=global
      link override ES: Cap=36500  SoCin=0.8  Pin=17300  Pout=-17300
      link override HP: P_HP=4800  C=5220  H=284
      link override PV: P_STCm=3100
      settings: SourceProductName=KIF2 Library
  HH177 : kif2/Household (Single Phase)  Ctag=CONS1  Atag=Signal  Itag=Irrad  Ttag=T_Amb  Wtag=Wind  HHtag=PQ_HH177  HHtagv=global  PVtag=PQ_PV177  PVtagv=global  EStag=PQ_ES177  EStagv=global  HPtag=PQ_HP177  HPtagv=global
      link override ES: Cap=9100  SoCin=0.2  Pin=5300  Pout=-5300
      link override HP: P_HP=2400  C=2655  H=140
      link override PV: P_STCm=800
      settings: SourceProductName=KIF2 Library
  HH178 : kif2/Household (Single Phase)  Ctag=CONS2  Atag=Signal  Itag=Irrad  Ttag=T_Amb  Wtag=Wind  HHtag=PQ_HH178  HHtagv=global  PVtag=PQ_PV178  PVtagv=global  EStag=PQ_ES178  EStagv=global  HPtag=PQ_HP178  HPtagv=global
      link override ES: Cap=13700  SoCin=0.3  Pin=7300  Pout=-7300
      link override HP: P_HP=3000  C=4950  H=141
      link override PV: P_STCm=1200
      settings: SourceProductName=KIF2 Library
  HH179 : kif2/Household (Single Phase)  Ctag=CONS3  Atag=Signal  Itag=Irrad  Ttag=T_Amb  Wtag=Wind  HHtag=PQ_HH179  HHtagv=global  PVtag=PQ_PV179  PVtagv=global  EStag=PQ_ES179  EStagv=global  HPtag=PQ_HP179  HPtagv=global
      link override ES: Cap=18300  SoCin=0.4  Pin=9300  Pout=-9300
      link override HP: P_HP=2500  C=2520  H=146
      link override PV: P_STCm=1500
      settings: SourceProductName=KIF2 Library
  HH18 : kif2/Household (Single Phase)  Ctag=CONS3  Atag=Signal  Itag=Irrad  Ttag=T_Amb  Wtag=Wind  HHtag=PQ_HH18  HHtagv=global  PVtag=PQ_PV18  PVtagv=global  EStag=PQ_ES18  EStagv=global  HPtag=PQ_HP18  HPtagv=global
      link override ES: Cap=18300  SoCin=0.4  Pin=9300  Pout=-9300
      link override HP: P_HP=2500  C=2520  H=146
      link override PV: P_STCm=1500
      settings: SourceProductName=KIF2 Library
  HH180 : kif2/Household (Single Phase)  Ctag=CONS4  Atag=Signal  Itag=Irrad  Ttag=T_Amb  Wtag=Wind  HHtag=PQ_HH180  HHtagv=global  PVtag=PQ_PV180  PVtagv=global  EStag=PQ_ES180  EStagv=global  HPtag=PQ_HP180  HPtagv=global
      link override ES: Cap=22800  Pin=11300  Pout=-11300
      link override HP: P_HP=3300  C=4635  H=176
      link override PV: P_STCm=1900
      settings: SourceProductName=KIF2 Library
  HH181 : kif2/Household (Single Phase)  Ctag=CONS5  Atag=Signal  Itag=Irrad  Ttag=T_Amb  Wtag=Wind  HHtag=PQ_HH181  HHtagv=global  PVtag=PQ_PV181  PVtagv=global  EStag=PQ_ES181  EStagv=global  HPtag=PQ_HP181  HPtagv=global
      link override ES: Cap=27400  SoCin=0.6  Pin=13300  Pout=-13300
      link override PV: P_STCm=2300
      settings: SourceProductName=KIF2 Library
  HH182 : kif2/Household (Single Phase)  Ctag=CONS6  Atag=Signal  Itag=Irrad  Ttag=T_Amb  Wtag=Wind  HHtag=PQ_HH182  HHtagv=global  PVtag=PQ_PV182  PVtagv=global  EStag=PQ_ES182  EStagv=global  HPtag=PQ_HP182  HPtagv=global
      link override ES: Cap=32000  SoCin=0.7  Pin=15300  Pout=-15300
      link override HP: P_HP=4200  C=4590  H=241
      settings: SourceProductName=KIF2 Library
  HH183 : kif2/Household  Ctag=CONS7  Atag=Signal  Itag=Irrad  Ttag=T_Amb  Wtag=Wind  HHtag=PQ_HH183  HHtagv=global  PVtag=PQ_PV183  PVtagv=global  EStag=PQ_ES183  EStagv=global  HPtag=PQ_HP183  HPtagv=global
      link override ES: Cap=36500  SoCin=0.8  Pin=17300  Pout=-17300
      link override HP: P_HP=4800  C=5220  H=284
      link override PV: P_STCm=3100
      settings: SourceProductName=KIF2 Library
  HH184 : kif2/Household (Single Phase)  Ctag=CONS1  Atag=Signal  Itag=Irrad  Ttag=T_Amb  Wtag=Wind  HHtag=PQ_HH184  HHtagv=global  PVtag=PQ_PV184  PVtagv=global  EStag=PQ_ES184  EStagv=global  HPtag=PQ_HP184  HPtagv=global
      link override ES: Cap=9100  SoCin=0.2  Pin=5300  Pout=-5300
      link override HP: P_HP=2400  C=2655  H=140
      link override PV: P_STCm=800
      settings: SourceProductName=KIF2 Library
  HH185 : kif2/Household (Single Phase)  Ctag=CONS2  Atag=Signal  Itag=Irrad  Ttag=T_Amb  Wtag=Wind  HHtag=PQ_HH185  HHtagv=global  PVtag=PQ_PV185  PVtagv=global  EStag=PQ_ES185  EStagv=global  HPtag=PQ_HP185  HPtagv=global
      link override ES: Cap=13700  SoCin=0.3  Pin=7300  Pout=-7300
      link override HP: P_HP=3000  C=4950  H=141
      link override PV: P_STCm=1200
      settings: SourceProductName=KIF2 Library
  HH186 : kif2/Household (Single Phase)  Ctag=CONS3  Atag=Signal  Itag=Irrad  Ttag=T_Amb  Wtag=Wind  HHtag=PQ_HH186  HHtagv=global  PVtag=PQ_PV186  PVtagv=global  EStag=PQ_ES186  EStagv=global  HPtag=PQ_HP186  HPtagv=global
      link override ES: Cap=18300  SoCin=0.4  Pin=9300  Pout=-9300
      link override HP: P_HP=2500  C=2520  H=146
      link override PV: P_STCm=1500
      settings: SourceProductName=KIF2 Library
  HH187 : kif2/Household (Single Phase)  Ctag=CONS4  Atag=Signal  Itag=Irrad  Ttag=T_Amb  Wtag=Wind  HHtag=PQ_HH187  HHtagv=global  PVtag=PQ_PV187  PVtagv=global  EStag=PQ_ES187  EStagv=global  HPtag=PQ_HP187  HPtagv=global
      link override ES: Cap=22800  Pin=11300  Pout=-11300
      link override HP: P_HP=3300  C=4635  H=176
      link override PV: P_STCm=1900
      settings: SourceProductName=KIF2 Library
  HH188 : kif2/Household (Single Phase)  Ctag=CONS5  Atag=Signal  Itag=Irrad  Ttag=T_Amb  Wtag=Wind  HHtag=PQ_HH188  HHtagv=global  PVtag=PQ_PV188  PVtagv=global  EStag=PQ_ES188  EStagv=global  HPtag=PQ_HP188  HPtagv=global
      link override ES: Cap=27400  SoCin=0.6  Pin=13300  Pout=-13300
      link override PV: P_STCm=2300
      settings: SourceProductName=KIF2 Library
  HH189 : kif2/Household (Single Phase)  Ctag=CONS6  Atag=Signal  Itag=Irrad  Ttag=T_Amb  Wtag=Wind  HHtag=PQ_HH189  HHtagv=global  PVtag=PQ_PV189  PVtagv=global  EStag=PQ_ES189  EStagv=global  HPtag=PQ_HP189  HPtagv=global
      link override ES: Cap=32000  SoCin=0.7  Pin=15300  Pout=-15300
      link override HP: P_HP=4200  C=4590  H=241
      settings: SourceProductName=KIF2 Library
  HH19 : kif2/Household (Single Phase)  Ctag=CONS4  Atag=Signal  Itag=Irrad  Ttag=T_Amb  Wtag=Wind  HHtag=PQ_HH19  HHtagv=global  PVtag=PQ_PV19  PVtagv=global  EStag=PQ_ES19  EStagv=global  HPtag=PQ_HP19  HPtagv=global
      link override ES: Cap=22800  Pin=11300  Pout=-11300
      link override HP: P_HP=3300  C=4635  H=176
      link override PV: P_STCm=1900
      settings: SourceProductName=KIF2 Library
  HH190 : kif2/Household  Ctag=CONS7  Atag=Signal  Itag=Irrad  Ttag=T_Amb  Wtag=Wind  HHtag=PQ_HH190  HHtagv=global  PVtag=PQ_PV190  PVtagv=global  EStag=PQ_ES190  EStagv=global  HPtag=PQ_HP190  HPtagv=global
      link override ES: Cap=36500  SoCin=0.8  Pin=17300  Pout=-17300
      link override HP: P_HP=4800  C=5220  H=284
      link override PV: P_STCm=3100
      settings: SourceProductName=KIF2 Library
  HH191 : kif2/Household (Single Phase)  Ctag=CONS1  Atag=Signal  Itag=Irrad  Ttag=T_Amb  Wtag=Wind  HHtag=PQ_HH191  HHtagv=global  PVtag=PQ_PV191  PVtagv=global  EStag=PQ_ES191  EStagv=global  HPtag=PQ_HP191  HPtagv=global
      link override ES: Cap=9100  SoCin=0.2  Pin=5300  Pout=-5300
      link override HP: P_HP=2400  C=2655  H=140
      link override PV: P_STCm=800
      settings: SourceProductName=KIF2 Library
  HH192 : kif2/Household (Single Phase)  Ctag=CONS2  Atag=Signal  Itag=Irrad  Ttag=T_Amb  Wtag=Wind  HHtag=PQ_HH192  HHtagv=global  PVtag=PQ_PV192  PVtagv=global  EStag=PQ_ES192  EStagv=global  HPtag=PQ_HP192  HPtagv=global
      link override ES: Cap=13700  SoCin=0.3  Pin=7300  Pout=-7300
      link override HP: P_HP=3000  C=4950  H=141
      link override PV: P_STCm=1200
      settings: SourceProductName=KIF2 Library
  HH193 : kif2/Household (Single Phase)  Ctag=CONS3  Atag=Signal  Itag=Irrad  Ttag=T_Amb  Wtag=Wind  HHtag=PQ_HH193  HHtagv=global  PVtag=PQ_PV193  PVtagv=global  EStag=PQ_ES193  EStagv=global  HPtag=PQ_HP193  HPtagv=global
      link override ES: Cap=18300  SoCin=0.4  Pin=9300  Pout=-9300
      link override HP: P_HP=2500  C=2520  H=146
      link override PV: P_STCm=1500
      settings: SourceProductName=KIF2 Library
  HH194 : kif2/Household (Single Phase)  Ctag=CONS4  Atag=Signal  Itag=Irrad  Ttag=T_Amb  Wtag=Wind  HHtag=PQ_HH194  HHtagv=global  PVtag=PQ_PV194  PVtagv=global  EStag=PQ_ES194  EStagv=global  HPtag=PQ_HP194  HPtagv=global
      link override ES: Cap=22800  Pin=11300  Pout=-11300
      link override HP: P_HP=3300  C=4635  H=176
      link override PV: P_STCm=1900
      settings: SourceProductName=KIF2 Library
  HH195 : kif2/Household (Single Phase)  Ctag=CONS5  Atag=Signal  Itag=Irrad  Ttag=T_Amb  Wtag=Wind  HHtag=PQ_HH195  HHtagv=global  PVtag=PQ_PV195  PVtagv=global  EStag=PQ_ES195  EStagv=global  HPtag=PQ_HP195  HPtagv=global
      link override ES: Cap=27400  SoCin=0.6  Pin=13300  Pout=-13300
      link override PV: P_STCm=2300
      settings: SourceProductName=KIF2 Library
  HH196 : kif2/Household (Single Phase)  Ctag=CONS6  Atag=Signal  Itag=Irrad  Ttag=T_Amb  Wtag=Wind  HHtag=PQ_HH196  HHtagv=global  PVtag=PQ_PV196  PVtagv=global  EStag=PQ_ES196  EStagv=global  HPtag=PQ_HP196  HPtagv=global
      link override ES: Cap=32000  SoCin=0.7  Pin=15300  Pout=-15300
      link override HP: P_HP=4200  C=4590  H=241
      settings: SourceProductName=KIF2 Library
  HH197 : kif2/Household  Ctag=CONS7  Atag=Signal  Itag=Irrad  Ttag=T_Amb  Wtag=Wind  HHtag=PQ_HH197  HHtagv=global  PVtag=PQ_PV197  PVtagv=global  EStag=PQ_ES197  EStagv=global  HPtag=PQ_HP197  HPtagv=global
      link override ES: Cap=36500  SoCin=0.8  Pin=17300  Pout=-17300
      link override HP: P_HP=4800  C=5220  H=284
      link override PV: P_STCm=3100
      settings: SourceProductName=KIF2 Library
  HH198 : kif2/Household (Single Phase)  Ctag=CONS1  Atag=Signal  Itag=Irrad  Ttag=T_Amb  Wtag=Wind  HHtag=PQ_HH198  HHtagv=global  PVtag=PQ_PV198  PVtagv=global  EStag=PQ_ES198  EStagv=global  HPtag=PQ_HP198  HPtagv=global
      link override ES: Cap=9100  SoCin=0.2  Pin=5300  Pout=-5300
      link override HP: P_HP=2400  C=2655  H=140
      link override PV: P_STCm=800
      settings: SourceProductName=KIF2 Library
  HH199 : kif2/Household (Single Phase)  Ctag=CONS2  Atag=Signal  Itag=Irrad  Ttag=T_Amb  Wtag=Wind  HHtag=PQ_HH199  HHtagv=global  PVtag=PQ_PV199  PVtagv=global  EStag=PQ_ES199  EStagv=global  HPtag=PQ_HP199  HPtagv=global
      link override ES: Cap=13700  SoCin=0.3  Pin=7300  Pout=-7300
      link override HP: P_HP=3000  C=4950  H=141
      link override PV: P_STCm=1200
      settings: SourceProductName=KIF2 Library
  HH2 : kif2/Household (Single Phase)  Ctag=CONS1  Atag=Signal  Itag=Irrad  Ttag=T_Amb  Wtag=Wind  HHtag=PQ_HH2  HHtagv=global  PVtag=PQ_PV2  PVtagv=global  EStag=PQ_ES2  EStagv=global  HPtag=PQ_HP2  HPtagv=global
      link override ES: Cap=9100  SoCin=0.2  Pin=5300  Pout=-5300
      link override HP: P_HP=2400  C=2655  H=140
      link override PV: P_STCm=800
      settings: SourceProductName=KIF2 Library
  HH20 : kif2/Household (Single Phase)  Ctag=CONS5  Atag=Signal  Itag=Irrad  Ttag=T_Amb  Wtag=Wind  HHtag=PQ_HH20  HHtagv=global  PVtag=PQ_PV20  PVtagv=global  EStag=PQ_ES20  EStagv=global  HPtag=PQ_HP20  HPtagv=global
      link override ES: Cap=27400  SoCin=0.6  Pin=13300  Pout=-13300
      link override PV: P_STCm=2300
      settings: SourceProductName=KIF2 Library
  HH200 : kif2/Household (Single Phase)  Ctag=CONS3  Atag=Signal  Itag=Irrad  Ttag=T_Amb  Wtag=Wind  HHtag=PQ_HH200  HHtagv=global  PVtag=PQ_PV200  PVtagv=global  EStag=PQ_ES200  EStagv=global  HPtag=PQ_HP200  HPtagv=global
      link override ES: Cap=18300  SoCin=0.4  Pin=9300  Pout=-9300
      link override HP: P_HP=2500  C=2520  H=146
      link override PV: P_STCm=1500
      settings: SourceProductName=KIF2 Library
  HH201 : kif2/Household  Ctag=CONS7  Atag=Signal  Itag=Irrad  Ttag=T_Amb  Wtag=Wind  HHtag=PQ_HH201  HHtagv=global  PVtag=PQ_PV201  PVtagv=global  EStag=PQ_ES201  EStagv=global  HPtag=PQ_HP201  HPtagv=global
      link override ES: Cap=36500  SoCin=0.8  Pin=17300  Pout=-17300
      link override HP: P_HP=4800  C=5220  H=284
      link override PV: P_STCm=3100
      settings: SourceProductName=KIF2 Library
  HH21 : kif2/Household (Single Phase)  Ctag=CONS6  Atag=Signal  Itag=Irrad  Ttag=T_Amb  Wtag=Wind  HHtag=PQ_HH21  HHtagv=global  PVtag=PQ_PV21  PVtagv=global  EStag=PQ_ES21  EStagv=global  HPtag=PQ_HP21  HPtagv=global
      link override ES: Cap=32000  SoCin=0.7  Pin=15300  Pout=-15300
      link override HP: P_HP=4200  C=4590  H=241
      settings: SourceProductName=KIF2 Library
  HH22 : kif2/Household  Ctag=CONS7  Atag=Signal  Itag=Irrad  Ttag=T_Amb  Wtag=Wind  HHtag=PQ_HH22  HHtagv=global  PVtag=PQ_PV22  PVtagv=global  EStag=PQ_ES22  EStagv=global  HPtag=PQ_HP22  HPtagv=global
      link override ES: Cap=36500  SoCin=0.8  Pin=17300  Pout=-17300
      link override HP: P_HP=4800  C=5220  H=284
      link override PV: P_STCm=3100
      settings: SourceProductName=KIF2 Library
  HH23 : kif2/Household (Single Phase)  Ctag=CONS1  Atag=Signal  Itag=Irrad  Ttag=T_Amb  Wtag=Wind  HHtag=PQ_HH23  HHtagv=global  PVtag=PQ_PV23  PVtagv=global  EStag=PQ_ES23  EStagv=global  HPtag=PQ_HP23  HPtagv=global
      link override ES: Cap=9100  SoCin=0.2  Pin=5300  Pout=-5300
      link override HP: P_HP=2400  C=2655  H=140
      link override PV: P_STCm=800
      settings: SourceProductName=KIF2 Library
  HH24 : kif2/Household (Single Phase)  Ctag=CONS2  Atag=Signal  Itag=Irrad  Ttag=T_Amb  Wtag=Wind  HHtag=PQ_HH24  HHtagv=global  PVtag=PQ_PV24  PVtagv=global  EStag=PQ_ES24  EStagv=global  HPtag=PQ_HP24  HPtagv=global
      link override ES: Cap=13700  SoCin=0.3  Pin=7300  Pout=-7300
      link override HP: P_HP=3000  C=4950  H=141
      link override PV: P_STCm=1200
      settings: SourceProductName=KIF2 Library
  HH25 : kif2/Household (Single Phase)  Ctag=CONS3  Atag=Signal  Itag=Irrad  Ttag=T_Amb  Wtag=Wind  HHtag=PQ_HH25  HHtagv=global  PVtag=PQ_PV25  PVtagv=global  EStag=PQ_ES25  EStagv=global  HPtag=PQ_HP25  HPtagv=global
      link override ES: Cap=18300  SoCin=0.4  Pin=9300  Pout=-9300
      link override HP: P_HP=2500  C=2520  H=146
      link override PV: P_STCm=1500
      settings: SourceProductName=KIF2 Library
  HH26 : kif2/Household (Single Phase)  Ctag=CONS4  Atag=Signal  Itag=Irrad  Ttag=T_Amb  Wtag=Wind  HHtag=PQ_HH26  HHtagv=global  PVtag=PQ_PV26  PVtagv=global  EStag=PQ_ES26  EStagv=global  HPtag=PQ_HP26  HPtagv=global
      link override ES: Cap=22800  Pin=11300  Pout=-11300
      link override HP: P_HP=3300  C=4635  H=176
      link override PV: P_STCm=1900
      settings: SourceProductName=KIF2 Library
  HH27 : kif2/Household (Single Phase)  Ctag=CONS5  Atag=Signal  Itag=Irrad  Ttag=T_Amb  Wtag=Wind  HHtag=PQ_HH27  HHtagv=global  PVtag=PQ_PV27  PVtagv=global  EStag=PQ_ES27  EStagv=global  HPtag=PQ_HP27  HPtagv=global
      link override ES: Cap=27400  SoCin=0.6  Pin=13300  Pout=-13300
      link override PV: P_STCm=2300
      settings: SourceProductName=KIF2 Library
  HH28 : kif2/Household (Single Phase)  Ctag=CONS6  Atag=Signal  Itag=Irrad  Ttag=T_Amb  Wtag=Wind  HHtag=PQ_HH28  HHtagv=global  PVtag=PQ_PV28  PVtagv=global  EStag=PQ_ES28  EStagv=global  HPtag=PQ_HP28  HPtagv=global
      link override ES: Cap=32000  SoCin=0.7  Pin=15300  Pout=-15300
      link override HP: P_HP=4200  C=4590  H=241
      settings: SourceProductName=KIF2 Library
  HH29 : kif2/Household  Ctag=CONS7  Atag=Signal  Itag=Irrad  Ttag=T_Amb  Wtag=Wind  HHtag=PQ_HH29  HHtagv=global  PVtag=PQ_PV29  PVtagv=global  EStag=PQ_ES29  EStagv=global  HPtag=PQ_HP29  HPtagv=global
      link override ES: Cap=36500  SoCin=0.8  Pin=17300  Pout=-17300
      link override HP: P_HP=4800  C=5220  H=284
      link override PV: P_STCm=3100
      settings: SourceProductName=KIF2 Library
  HH3 : kif2/Household (Single Phase)  Ctag=CONS2  Atag=Signal  Itag=Irrad  Ttag=T_Amb  Wtag=Wind  HHtag=PQ_HH3  HHtagv=global  PVtag=PQ_PV3  PVtagv=global  EStag=PQ_ES3  EStagv=global  HPtag=PQ_HP3  HPtagv=global
      link override ES: Cap=13700  SoCin=0.3  Pin=7300  Pout=-7300
      link override HP: P_HP=3000  C=4950  H=141
      link override PV: P_STCm=1200
      settings: SourceProductName=KIF2 Library
  HH30 : kif2/Household (Single Phase)  Ctag=CONS1  Atag=Signal  Itag=Irrad  Ttag=T_Amb  Wtag=Wind  HHtag=PQ_HH30  HHtagv=global  PVtag=PQ_PV30  PVtagv=global  EStag=PQ_ES30  EStagv=global  HPtag=PQ_HP30  HPtagv=global
      link override ES: Cap=9100  SoCin=0.2  Pin=5300  Pout=-5300
      link override HP: P_HP=2400  C=2655  H=140
      link override PV: P_STCm=800
      settings: SourceProductName=KIF2 Library
  HH31 : kif2/Household (Single Phase)  Ctag=CONS2  Atag=Signal  Itag=Irrad  Ttag=T_Amb  Wtag=Wind  HHtag=PQ_HH31  HHtagv=global  PVtag=PQ_PV31  PVtagv=global  EStag=PQ_ES31  EStagv=global  HPtag=PQ_HP31  HPtagv=global
      link override ES: Cap=13700  SoCin=0.3  Pin=7300  Pout=-7300
      link override HP: P_HP=3000  C=4950  H=141
      link override PV: P_STCm=1200
      settings: SourceProductName=KIF2 Library
  HH32 : kif2/Household (Single Phase)  Ctag=CONS3  Atag=Signal  Itag=Irrad  Ttag=T_Amb  Wtag=Wind  HHtag=PQ_HH32  HHtagv=global  PVtag=PQ_PV32  PVtagv=global  EStag=PQ_ES32  EStagv=global  HPtag=PQ_HP32  HPtagv=global
      link override ES: Cap=18300  SoCin=0.4  Pin=9300  Pout=-9300
      link override HP: P_HP=2500  C=2520  H=146
      link override PV: P_STCm=1500
      settings: SourceProductName=KIF2 Library
  HH33 : kif2/Household (Single Phase)  Ctag=CONS4  Atag=Signal  Itag=Irrad  Ttag=T_Amb  Wtag=Wind  HHtag=PQ_HH33  HHtagv=global  PVtag=PQ_PV33  PVtagv=global  EStag=PQ_ES33  EStagv=global  HPtag=PQ_HP33  HPtagv=global
      link override ES: Cap=22800  Pin=11300  Pout=-11300
      link override HP: P_HP=3300  C=4635  H=176
      link override PV: P_STCm=1900
      settings: SourceProductName=KIF2 Library
  HH34 : kif2/Household (Single Phase)  Ctag=CONS5  Atag=Signal  Itag=Irrad  Ttag=T_Amb  Wtag=Wind  HHtag=PQ_HH34  HHtagv=global  PVtag=PQ_PV34  PVtagv=global  EStag=PQ_ES34  EStagv=global  HPtag=PQ_HP34  HPtagv=global
      link override ES: Cap=27400  SoCin=0.6  Pin=13300  Pout=-13300
      link override PV: P_STCm=2300
      settings: SourceProductName=KIF2 Library
  HH35 : kif2/Household (Single Phase)  Ctag=CONS6  Atag=Signal  Itag=Irrad  Ttag=T_Amb  Wtag=Wind  HHtag=PQ_HH35  HHtagv=global  PVtag=PQ_PV35  PVtagv=global  EStag=PQ_ES35  EStagv=global  HPtag=PQ_HP35  HPtagv=global
      link override ES: Cap=32000  SoCin=0.7  Pin=15300  Pout=-15300
      link override HP: P_HP=4200  C=4590  H=241
      settings: SourceProductName=KIF2 Library
  HH36 : kif2/Household  Ctag=CONS7  Atag=Signal  Itag=Irrad  Ttag=T_Amb  Wtag=Wind  HHtag=PQ_HH36  HHtagv=global  PVtag=PQ_PV36  PVtagv=global  EStag=PQ_ES36  EStagv=global  HPtag=PQ_HP36  HPtagv=global
      link override ES: Cap=36500  SoCin=0.8  Pin=17300  Pout=-17300
      link override HP: P_HP=4800  C=5220  H=284
      link override PV: P_STCm=3100
      settings: SourceProductName=KIF2 Library
  HH37 : kif2/Household (Single Phase)  Ctag=CONS1  Atag=Signal  Itag=Irrad  Ttag=T_Amb  Wtag=Wind  HHtag=PQ_HH37  HHtagv=global  PVtag=PQ_PV37  PVtagv=global  EStag=PQ_ES37  EStagv=global  HPtag=PQ_HP37  HPtagv=global
      link override ES: Cap=9100  SoCin=0.2  Pin=5300  Pout=-5300
      link override HP: P_HP=2400  C=2655  H=140
      link override PV: P_STCm=800
      settings: SourceProductName=KIF2 Library
  HH38 : kif2/Household (Single Phase)  Ctag=CONS2  Atag=Signal  Itag=Irrad  Ttag=T_Amb  Wtag=Wind  HHtag=PQ_HH38  HHtagv=global  PVtag=PQ_PV38  PVtagv=global  EStag=PQ_ES38  EStagv=global  HPtag=PQ_HP38  HPtagv=global
      link override ES: Cap=13700  SoCin=0.3  Pin=7300  Pout=-7300
      link override HP: P_HP=3000  C=4950  H=141
      link override PV: P_STCm=1200
      settings: SourceProductName=KIF2 Library
  HH39 : kif2/Household (Single Phase)  Ctag=CONS3  Atag=Signal  Itag=Irrad  Ttag=T_Amb  Wtag=Wind  HHtag=PQ_HH39  HHtagv=global  PVtag=PQ_PV39  PVtagv=global  EStag=PQ_ES39  EStagv=global  HPtag=PQ_HP39  HPtagv=global
      link override ES: Cap=18300  SoCin=0.4  Pin=9300  Pout=-9300
      link override HP: P_HP=2500  C=2520  H=146
      link override PV: P_STCm=1500
      settings: SourceProductName=KIF2 Library
  HH4 : kif2/Household (Single Phase)  Ctag=CONS3  Atag=Signal  Itag=Irrad  Ttag=T_Amb  Wtag=Wind  HHtag=PQ_HH4  HHtagv=global  PVtag=PQ_PV4  PVtagv=global  EStag=PQ_ES4  EStagv=global  HPtag=PQ_HP4  HPtagv=global
      link override ES: Cap=18300  SoCin=0.4  Pin=9300  Pout=-9300
      link override HP: P_HP=2500  C=2520  H=146
      link override PV: P_STCm=1500
      settings: SourceProductName=KIF2 Library
  HH40 : kif2/Household (Single Phase)  Ctag=CONS4  Atag=Signal  Itag=Irrad  Ttag=T_Amb  Wtag=Wind  HHtag=PQ_HH40  HHtagv=global  PVtag=PQ_PV40  PVtagv=global  EStag=PQ_ES40  EStagv=global  HPtag=PQ_HP40  HPtagv=global
      link override ES: Cap=22800  Pin=11300  Pout=-11300
      link override HP: P_HP=3300  C=4635  H=176
      link override PV: P_STCm=1900
      settings: SourceProductName=KIF2 Library
  HH41 : kif2/Household (Single Phase)  Ctag=CONS5  Atag=Signal  Itag=Irrad  Ttag=T_Amb  Wtag=Wind  HHtag=PQ_HH41  HHtagv=global  PVtag=PQ_PV41  PVtagv=global  EStag=PQ_ES41  EStagv=global  HPtag=PQ_HP41  HPtagv=global
      link override ES: Cap=27400  SoCin=0.6  Pin=13300  Pout=-13300
      link override PV: P_STCm=2300
      settings: SourceProductName=KIF2 Library
  HH42 : kif2/Household (Single Phase)  Ctag=CONS6  Atag=Signal  Itag=Irrad  Ttag=T_Amb  Wtag=Wind  HHtag=PQ_HH42  HHtagv=global  PVtag=PQ_PV42  PVtagv=global  EStag=PQ_ES42  EStagv=global  HPtag=PQ_HP42  HPtagv=global
      link override ES: Cap=32000  SoCin=0.7  Pin=15300  Pout=-15300
      link override HP: P_HP=4200  C=4590  H=241
      settings: SourceProductName=KIF2 Library
  HH43 : kif2/Household  Ctag=CONS7  Atag=Signal  Itag=Irrad  Ttag=T_Amb  Wtag=Wind  HHtag=PQ_HH43  HHtagv=global  PVtag=PQ_PV43  PVtagv=global  EStag=PQ_ES43  EStagv=global  HPtag=PQ_HP43  HPtagv=global
      link override ES: Cap=36500  SoCin=0.8  Pin=17300  Pout=-17300
      link override HP: P_HP=4800  C=5220  H=284
      link override PV: P_STCm=3100
      settings: SourceProductName=KIF2 Library
  HH44 : kif2/Household (Single Phase)  Ctag=CONS1  Atag=Signal  Itag=Irrad  Ttag=T_Amb  Wtag=Wind  HHtag=PQ_HH44  HHtagv=global  PVtag=PQ_PV44  PVtagv=global  EStag=PQ_ES44  EStagv=global  HPtag=PQ_HP44  HPtagv=global
      link override ES: Cap=9100  SoCin=0.2  Pin=5300  Pout=-5300
      link override HP: P_HP=2400  C=2655  H=140
      link override PV: P_STCm=800
      settings: SourceProductName=KIF2 Library
  HH45 : kif2/Household (Single Phase)  Ctag=CONS2  Atag=Signal  Itag=Irrad  Ttag=T_Amb  Wtag=Wind  HHtag=PQ_HH45  HHtagv=global  PVtag=PQ_PV45  PVtagv=global  EStag=PQ_ES45  EStagv=global  HPtag=PQ_HP45  HPtagv=global
      link override ES: Cap=13700  SoCin=0.3  Pin=7300  Pout=-7300
      link override HP: P_HP=3000  C=4950  H=141
      link override PV: P_STCm=1200
      settings: SourceProductName=KIF2 Library
  HH46 : kif2/Household (Single Phase)  Ctag=CONS3  Atag=Signal  Itag=Irrad  Ttag=T_Amb  Wtag=Wind  HHtag=PQ_HH46  HHtagv=global  PVtag=PQ_PV46  PVtagv=global  EStag=PQ_ES46  EStagv=global  HPtag=PQ_HP46  HPtagv=global
      link override ES: Cap=18300  SoCin=0.4  Pin=9300  Pout=-9300
      link override HP: P_HP=2500  C=2520  H=146
      link override PV: P_STCm=1500
      settings: SourceProductName=KIF2 Library
  HH47 : kif2/Household (Single Phase)  Ctag=CONS4  Atag=Signal  Itag=Irrad  Ttag=T_Amb  Wtag=Wind  HHtag=PQ_HH47  HHtagv=global  PVtag=PQ_PV47  PVtagv=global  EStag=PQ_ES47  EStagv=global  HPtag=PQ_HP47  HPtagv=global
      link override ES: Cap=22800  Pin=11300  Pout=-11300
      link override HP: P_HP=3300  C=4635  H=176
      link override PV: P_STCm=1900
      settings: SourceProductName=KIF2 Library
  HH48 : kif2/Household (Single Phase)  Ctag=CONS5  Atag=Signal  Itag=Irrad  Ttag=T_Amb  Wtag=Wind  HHtag=PQ_HH48  HHtagv=global  PVtag=PQ_PV48  PVtagv=global  EStag=PQ_ES48  EStagv=global  HPtag=PQ_HP48  HPtagv=global
      link override ES: Cap=27400  SoCin=0.6  Pin=13300  Pout=-13300
      link override PV: P_STCm=2300
      settings: SourceProductName=KIF2 Library
  HH49 : kif2/Household (Single Phase)  Ctag=CONS6  Atag=Signal  Itag=Irrad  Ttag=T_Amb  Wtag=Wind  HHtag=PQ_HH49  HHtagv=global  PVtag=PQ_PV49  PVtagv=global  EStag=PQ_ES49  EStagv=global  HPtag=PQ_HP49  HPtagv=global
      link override ES: Cap=32000  SoCin=0.7  Pin=15300  Pout=-15300
      link override HP: P_HP=4200  C=4590  H=241
      settings: SourceProductName=KIF2 Library
  HH5 : kif2/Household (Single Phase)  Ctag=CONS4  Atag=Signal  Itag=Irrad  Ttag=T_Amb  Wtag=Wind  HHtag=PQ_HH5  HHtagv=global  PVtag=PQ_PV5  PVtagv=global  EStag=PQ_ES5  EStagv=global  HPtag=PQ_HP5  HPtagv=global
      link override ES: Cap=22800  Pin=11300  Pout=-11300
      link override HP: P_HP=3300  C=4635  H=176
      link override PV: P_STCm=1900
      settings: SourceProductName=KIF2 Library
  HH50 : kif2/Household  Ctag=CONS7  Atag=Signal  Itag=Irrad  Ttag=T_Amb  Wtag=Wind  HHtag=PQ_HH50  HHtagv=global  PVtag=PQ_PV50  PVtagv=global  EStag=PQ_ES50  EStagv=global  HPtag=PQ_HP50  HPtagv=global
      link override ES: Cap=36500  SoCin=0.8  Pin=17300  Pout=-17300
      link override HP: P_HP=4800  C=5220  H=284
      link override PV: P_STCm=3100
      settings: SourceProductName=KIF2 Library
  HH51 : kif2/Household (Single Phase)  Ctag=CONS1  Atag=Signal  Itag=Irrad  Ttag=T_Amb  Wtag=Wind  HHtag=PQ_HH51  HHtagv=global  PVtag=PQ_PV51  PVtagv=global  EStag=PQ_ES51  EStagv=global  HPtag=PQ_HP51  HPtagv=global
      link override ES: Cap=9100  SoCin=0.2  Pin=5300  Pout=-5300
      link override HP: P_HP=2400  C=2655  H=140
      link override PV: P_STCm=800
      settings: SourceProductName=KIF2 Library
  HH52 : kif2/Household (Single Phase)  Ctag=CONS2  Atag=Signal  Itag=Irrad  Ttag=T_Amb  Wtag=Wind  HHtag=PQ_HH52  HHtagv=global  PVtag=PQ_PV52  PVtagv=global  EStag=PQ_ES52  EStagv=global  HPtag=PQ_HP52  HPtagv=global
      link override ES: Cap=13700  SoCin=0.3  Pin=7300  Pout=-7300
      link override HP: P_HP=3000  C=4950  H=141
      link override PV: P_STCm=1200
      settings: SourceProductName=KIF2 Library
  HH53 : kif2/Household (Single Phase)  Ctag=CONS3  Atag=Signal  Itag=Irrad  Ttag=T_Amb  Wtag=Wind  HHtag=PQ_HH53  HHtagv=global  PVtag=PQ_PV53  PVtagv=global  EStag=PQ_ES53  EStagv=global  HPtag=PQ_HP53  HPtagv=global
      link override ES: Cap=18300  SoCin=0.4  Pin=9300  Pout=-9300
      link override HP: P_HP=2500  C=2520  H=146
      link override PV: P_STCm=1500
      settings: SourceProductName=KIF2 Library
  HH54 : kif2/Household (Single Phase)  Ctag=CONS4  Atag=Signal  Itag=Irrad  Ttag=T_Amb  Wtag=Wind  HHtag=PQ_HH54  HHtagv=global  PVtag=PQ_PV54  PVtagv=global  EStag=PQ_ES54  EStagv=global  HPtag=PQ_HP54  HPtagv=global
      link override ES: Cap=22800  Pin=11300  Pout=-11300
      link override HP: P_HP=3300  C=4635  H=176
      link override PV: P_STCm=1900
      settings: SourceProductName=KIF2 Library
  HH55 : kif2/Household (Single Phase)  Ctag=CONS5  Atag=Signal  Itag=Irrad  Ttag=T_Amb  Wtag=Wind  HHtag=PQ_HH55  HHtagv=global  PVtag=PQ_PV55  PVtagv=global  EStag=PQ_ES55  EStagv=global  HPtag=PQ_HP55  HPtagv=global
      link override ES: Cap=27400  SoCin=0.6  Pin=13300  Pout=-13300
      link override PV: P_STCm=2300
      settings: SourceProductName=KIF2 Library
  HH56 : kif2/Household (Single Phase)  Ctag=CONS6  Atag=Signal  Itag=Irrad  Ttag=T_Amb  Wtag=Wind  HHtag=PQ_HH56  HHtagv=global  PVtag=PQ_PV56  PVtagv=global  EStag=PQ_ES56  EStagv=global  HPtag=PQ_HP56  HPtagv=global
      link override ES: Cap=32000  SoCin=0.7  Pin=15300  Pout=-15300
      link override HP: P_HP=4200  C=4590  H=241
      settings: SourceProductName=KIF2 Library
  HH57 : kif2/Household  Ctag=CONS7  Atag=Signal  Itag=Irrad  Ttag=T_Amb  Wtag=Wind  HHtag=PQ_HH57  HHtagv=global  PVtag=PQ_PV57  PVtagv=global  EStag=PQ_ES57  EStagv=global  HPtag=PQ_HP57  HPtagv=global
      link override ES: Cap=36500  SoCin=0.8  Pin=17300  Pout=-17300
      link override HP: P_HP=4800  C=5220  H=284
      link override PV: P_STCm=3100
      settings: SourceProductName=KIF2 Library
  HH58 : kif2/Household (Single Phase)  Ctag=CONS1  Atag=Signal  Itag=Irrad  Ttag=T_Amb  Wtag=Wind  HHtag=PQ_HH58  HHtagv=global  PVtag=PQ_PV58  PVtagv=global  EStag=PQ_ES58  EStagv=global  HPtag=PQ_HP58  HPtagv=global
      link override ES: Cap=9100  SoCin=0.2  Pin=5300  Pout=-5300
      link override HP: P_HP=2400  C=2655  H=140
      link override PV: P_STCm=800
      settings: SourceProductName=KIF2 Library
  HH59 : kif2/Household (Single Phase)  Ctag=CONS2  Atag=Signal  Itag=Irrad  Ttag=T_Amb  Wtag=Wind  HHtag=PQ_HH59  HHtagv=global  PVtag=PQ_PV59  PVtagv=global  EStag=PQ_ES59  EStagv=global  HPtag=PQ_HP59  HPtagv=global
      link override ES: Cap=13700  SoCin=0.3  Pin=7300  Pout=-7300
      link override HP: P_HP=3000  C=4950  H=141
      link override PV: P_STCm=1200
      settings: SourceProductName=KIF2 Library
  HH6 : kif2/Household (Single Phase)  Ctag=CONS5  Atag=Signal  Itag=Irrad  Ttag=T_Amb  Wtag=Wind  HHtag=PQ_HH6  HHtagv=global  PVtag=PQ_PV6  PVtagv=global  EStag=PQ_ES6  EStagv=global  HPtag=PQ_HP6  HPtagv=global
      link override ES: Cap=27400  SoCin=0.6  Pin=13300  Pout=-13300
      link override PV: P_STCm=2300
      settings: SourceProductName=KIF2 Library
  HH60 : kif2/Household (Single Phase)  Ctag=CONS3  Atag=Signal  Itag=Irrad  Ttag=T_Amb  Wtag=Wind  HHtag=PQ_HH60  HHtagv=global  PVtag=PQ_PV60  PVtagv=global  EStag=PQ_ES60  EStagv=global  HPtag=PQ_HP60  HPtagv=global
      link override ES: Cap=18300  SoCin=0.4  Pin=9300  Pout=-9300
      link override HP: P_HP=2500  C=2520  H=146
      link override PV: P_STCm=1500
      settings: SourceProductName=KIF2 Library
  HH61 : kif2/Household (Single Phase)  Ctag=CONS4  Atag=Signal  Itag=Irrad  Ttag=T_Amb  Wtag=Wind  HHtag=PQ_HH61  HHtagv=global  PVtag=PQ_PV61  PVtagv=global  EStag=PQ_ES61  EStagv=global  HPtag=PQ_HP61  HPtagv=global
      link override ES: Cap=22800  Pin=11300  Pout=-11300
      link override HP: P_HP=3300  C=4635  H=176
      link override PV: P_STCm=1900
      settings: SourceProductName=KIF2 Library
  HH62 : kif2/Household (Single Phase)  Ctag=CONS5  Atag=Signal  Itag=Irrad  Ttag=T_Amb  Wtag=Wind  HHtag=PQ_HH62  HHtagv=global  PVtag=PQ_PV62  PVtagv=global  EStag=PQ_ES62  EStagv=global  HPtag=PQ_HP62  HPtagv=global
      link override ES: Cap=27400  SoCin=0.6  Pin=13300  Pout=-13300
      link override PV: P_STCm=2300
      settings: SourceProductName=KIF2 Library
  HH63 : kif2/Household (Single Phase)  Ctag=CONS6  Atag=Signal  Itag=Irrad  Ttag=T_Amb  Wtag=Wind  HHtag=PQ_HH63  HHtagv=global  PVtag=PQ_PV63  PVtagv=global  EStag=PQ_ES63  EStagv=global  HPtag=PQ_HP63  HPtagv=global
      link override ES: Cap=32000  SoCin=0.7  Pin=15300  Pout=-15300
      link override HP: P_HP=4200  C=4590  H=241
      settings: SourceProductName=KIF2 Library
  HH64 : kif2/Household  Ctag=CONS7  Atag=Signal  Itag=Irrad  Ttag=T_Amb  Wtag=Wind  HHtag=PQ_HH64  HHtagv=global  PVtag=PQ_PV64  PVtagv=global  EStag=PQ_ES64  EStagv=global  HPtag=PQ_HP64  HPtagv=global
      link override ES: Cap=36500  SoCin=0.8  Pin=17300  Pout=-17300
      link override HP: P_HP=4800  C=5220  H=284
      link override PV: P_STCm=3100
      settings: SourceProductName=KIF2 Library
  HH65 : kif2/Household (Single Phase)  Ctag=CONS1  Atag=Signal  Itag=Irrad  Ttag=T_Amb  Wtag=Wind  HHtag=PQ_HH65  HHtagv=global  PVtag=PQ_PV65  PVtagv=global  EStag=PQ_ES65  EStagv=global  HPtag=PQ_HP65  HPtagv=global
      link override ES: Cap=9100  SoCin=0.2  Pin=5300  Pout=-5300
      link override HP: P_HP=2400  C=2655  H=140
      link override PV: P_STCm=800
      settings: SourceProductName=KIF2 Library
  HH66 : kif2/Household (Single Phase)  Ctag=CONS2  Atag=Signal  Itag=Irrad  Ttag=T_Amb  Wtag=Wind  HHtag=PQ_HH66  HHtagv=global  PVtag=PQ_PV66  PVtagv=global  EStag=PQ_ES66  EStagv=global  HPtag=PQ_HP66  HPtagv=global
      link override ES: Cap=13700  SoCin=0.3  Pin=7300  Pout=-7300
      link override HP: P_HP=3000  C=4950  H=141
      link override PV: P_STCm=1200
      settings: SourceProductName=KIF2 Library
  HH67 : kif2/Household (Single Phase)  Ctag=CONS3  Atag=Signal  Itag=Irrad  Ttag=T_Amb  Wtag=Wind  HHtag=PQ_HH67  HHtagv=global  PVtag=PQ_PV67  PVtagv=global  EStag=PQ_ES67  EStagv=global  HPtag=PQ_HP67  HPtagv=global
      link override ES: Cap=18300  SoCin=0.4  Pin=9300  Pout=-9300
      link override HP: P_HP=2500  C=2520  H=146
      link override PV: P_STCm=1500
      settings: SourceProductName=KIF2 Library
  HH68 : kif2/Household (Single Phase)  Ctag=CONS4  Atag=Signal  Itag=Irrad  Ttag=T_Amb  Wtag=Wind  HHtag=PQ_HH68  HHtagv=global  PVtag=PQ_PV68  PVtagv=global  EStag=PQ_ES68  EStagv=global  HPtag=PQ_HP68  HPtagv=global
      link override ES: Cap=22800  Pin=11300  Pout=-11300
      link override HP: P_HP=3300  C=4635  H=176
      link override PV: P_STCm=1900
      settings: SourceProductName=KIF2 Library
  HH69 : kif2/Household (Single Phase)  Ctag=CONS5  Atag=Signal  Itag=Irrad  Ttag=T_Amb  Wtag=Wind  HHtag=PQ_HH69  HHtagv=global  PVtag=PQ_PV69  PVtagv=global  EStag=PQ_ES69  EStagv=global  HPtag=PQ_HP69  HPtagv=global
      link override ES: Cap=27400  SoCin=0.6  Pin=13300  Pout=-13300
      link override PV: P_STCm=2300
      settings: SourceProductName=KIF2 Library
  HH7 : kif2/Household (Single Phase)  Ctag=CONS6  Atag=Signal  Itag=Irrad  Ttag=T_Amb  Wtag=Wind  HHtag=PQ_HH7  HHtagv=global  PVtag=PQ_PV7  PVtagv=global  EStag=PQ_ES7  EStagv=global  HPtag=PQ_HP7  HPtagv=global
      link override ES: Cap=32000  SoCin=0.7  Pin=15300  Pout=-15300
      link override HP: P_HP=4200  C=4590  H=241
      settings: SourceProductName=KIF2 Library
  HH70 : kif2/Household (Single Phase)  Ctag=CONS6  Atag=Signal  Itag=Irrad  Ttag=T_Amb  Wtag=Wind  HHtag=PQ_HH70  HHtagv=global  PVtag=PQ_PV70  PVtagv=global  EStag=PQ_ES70  EStagv=global  HPtag=PQ_HP70  HPtagv=global
      link override ES: Cap=32000  SoCin=0.7  Pin=15300  Pout=-15300
      link override HP: P_HP=4200  C=4590  H=241
      settings: SourceProductName=KIF2 Library
  HH71 : kif2/Household  Ctag=CONS7  Atag=Signal  Itag=Irrad  Ttag=T_Amb  Wtag=Wind  HHtag=PQ_HH71  HHtagv=global  PVtag=PQ_PV71  PVtagv=global  EStag=PQ_ES71  EStagv=global  HPtag=PQ_HP71  HPtagv=global
      link override ES: Cap=36500  SoCin=0.8  Pin=17300  Pout=-17300
      link override HP: P_HP=4800  C=5220  H=284
      link override PV: P_STCm=3100
      settings: SourceProductName=KIF2 Library
  HH72 : kif2/Household (Single Phase)  Ctag=CONS1  Atag=Signal  Itag=Irrad  Ttag=T_Amb  Wtag=Wind  HHtag=PQ_HH72  HHtagv=global  PVtag=PQ_PV72  PVtagv=global  EStag=PQ_ES72  EStagv=global  HPtag=PQ_HP72  HPtagv=global
      link override ES: Cap=9100  SoCin=0.2  Pin=5300  Pout=-5300
      link override HP: P_HP=2400  C=2655  H=140
      link override PV: P_STCm=800
      settings: SourceProductName=KIF2 Library
  HH73 : kif2/Household (Single Phase)  Ctag=CONS2  Atag=Signal  Itag=Irrad  Ttag=T_Amb  Wtag=Wind  HHtag=PQ_HH73  HHtagv=global  PVtag=PQ_PV73  PVtagv=global  EStag=PQ_ES73  EStagv=global  HPtag=PQ_HP73  HPtagv=global
      link override ES: Cap=13700  SoCin=0.3  Pin=7300  Pout=-7300
      link override HP: P_HP=3000  C=4950  H=141
      link override PV: P_STCm=1200
      settings: SourceProductName=KIF2 Library
  HH74 : kif2/Household (Single Phase)  Ctag=CONS3  Atag=Signal  Itag=Irrad  Ttag=T_Amb  Wtag=Wind  HHtag=PQ_HH74  HHtagv=global  PVtag=PQ_PV74  PVtagv=global  EStag=PQ_ES74  EStagv=global  HPtag=PQ_HP74  HPtagv=global
      link override ES: Cap=18300  SoCin=0.4  Pin=9300  Pout=-9300
      link override HP: P_HP=2500  C=2520  H=146
      link override PV: P_STCm=1500
      settings: SourceProductName=KIF2 Library
  HH75 : kif2/Household (Single Phase)  Ctag=CONS4  Atag=Signal  Itag=Irrad  Ttag=T_Amb  Wtag=Wind  HHtag=PQ_HH75  HHtagv=global  PVtag=PQ_PV75  PVtagv=global  EStag=PQ_ES75  EStagv=global  HPtag=PQ_HP75  HPtagv=global
      link override ES: Cap=22800  Pin=11300  Pout=-11300
      link override HP: P_HP=3300  C=4635  H=176
      link override PV: P_STCm=1900
      settings: SourceProductName=KIF2 Library
  HH76 : kif2/Household (Single Phase)  Ctag=CONS5  Atag=Signal  Itag=Irrad  Ttag=T_Amb  Wtag=Wind  HHtag=PQ_HH76  HHtagv=global  PVtag=PQ_PV76  PVtagv=global  EStag=PQ_ES76  EStagv=global  HPtag=PQ_HP76  HPtagv=global
      link override ES: Cap=27400  SoCin=0.6  Pin=13300  Pout=-13300
      link override PV: P_STCm=2300
      settings: SourceProductName=KIF2 Library
  HH77 : kif2/Household (Single Phase)  Ctag=CONS6  Atag=Signal  Itag=Irrad  Ttag=T_Amb  Wtag=Wind  HHtag=PQ_HH77  HHtagv=global  PVtag=PQ_PV77  PVtagv=global  EStag=PQ_ES77  EStagv=global  HPtag=PQ_HP77  HPtagv=global
      link override ES: Cap=32000  SoCin=0.7  Pin=15300  Pout=-15300
      link override HP: P_HP=4200  C=4590  H=241
      settings: SourceProductName=KIF2 Library
  HH78 : kif2/Household  Ctag=CONS7  Atag=Signal  Itag=Irrad  Ttag=T_Amb  Wtag=Wind  HHtag=PQ_HH78  HHtagv=global  PVtag=PQ_PV78  PVtagv=global  EStag=PQ_ES78  EStagv=global  HPtag=PQ_HP78  HPtagv=global
      link override ES: Cap=36500  SoCin=0.8  Pin=17300  Pout=-17300
      link override HP: P_HP=4800  C=5220  H=284
      link override PV: P_STCm=3100
      settings: SourceProductName=KIF2 Library
  HH79 : kif2/Household (Single Phase)  Ctag=CONS1  Atag=Signal  Itag=Irrad  Ttag=T_Amb  Wtag=Wind  HHtag=PQ_HH79  HHtagv=global  PVtag=PQ_PV79  PVtagv=global  EStag=PQ_ES79  EStagv=global  HPtag=PQ_HP79  HPtagv=global
      link override ES: Cap=9100  SoCin=0.2  Pin=5300  Pout=-5300
      link override HP: P_HP=2400  C=2655  H=140
      link override PV: P_STCm=800
      settings: SourceProductName=KIF2 Library
  HH8 : kif2/Household  Ctag=CONS7  Atag=Signal  Itag=Irrad  Ttag=T_Amb  Wtag=Wind  HHtag=PQ_HH8  HHtagv=global  PVtag=PQ_PV8  PVtagv=global  EStag=PQ_ES8  EStagv=global  HPtag=PQ_HP8  HPtagv=global
      link override ES: Cap=36500  SoCin=0.8  Pin=17300  Pout=-17300
      link override HP: P_HP=4800  C=5220  H=284
      link override PV: P_STCm=3100
      settings: SourceProductName=KIF2 Library
  HH80 : kif2/Household (Single Phase)  Ctag=CONS2  Atag=Signal  Itag=Irrad  Ttag=T_Amb  Wtag=Wind  HHtag=PQ_HH80  HHtagv=global  PVtag=PQ_PV80  PVtagv=global  EStag=PQ_ES80  EStagv=global  HPtag=PQ_HP80  HPtagv=global
      link override ES: Cap=13700  SoCin=0.3  Pin=7300  Pout=-7300
      link override HP: P_HP=3000  C=4950  H=141
      link override PV: P_STCm=1200
      settings: SourceProductName=KIF2 Library
  HH81 : kif2/Household (Single Phase)  Ctag=CONS3  Atag=Signal  Itag=Irrad  Ttag=T_Amb  Wtag=Wind  HHtag=PQ_HH81  HHtagv=global  PVtag=PQ_PV81  PVtagv=global  EStag=PQ_ES81  EStagv=global  HPtag=PQ_HP81  HPtagv=global
      link override ES: Cap=18300  SoCin=0.4  Pin=9300  Pout=-9300
      link override HP: P_HP=2500  C=2520  H=146
      link override PV: P_STCm=1500
      settings: SourceProductName=KIF2 Library
  HH82 : kif2/Household (Single Phase)  Ctag=CONS4  Atag=Signal  Itag=Irrad  Ttag=T_Amb  Wtag=Wind  HHtag=PQ_HH82  HHtagv=global  PVtag=PQ_PV82  PVtagv=global  EStag=PQ_ES82  EStagv=global  HPtag=PQ_HP82  HPtagv=global
      link override ES: Cap=22800  Pin=11300  Pout=-11300
      link override HP: P_HP=3300  C=4635  H=176
      link override PV: P_STCm=1900
      settings: SourceProductName=KIF2 Library
  HH83 : kif2/Household (Single Phase)  Ctag=CONS5  Atag=Signal  Itag=Irrad  Ttag=T_Amb  Wtag=Wind  HHtag=PQ_HH83  HHtagv=global  PVtag=PQ_PV83  PVtagv=global  EStag=PQ_ES83  EStagv=global  HPtag=PQ_HP83  HPtagv=global
      link override ES: Cap=27400  SoCin=0.6  Pin=13300  Pout=-13300
      link override PV: P_STCm=2300
      settings: SourceProductName=KIF2 Library
  HH84 : kif2/Household (Single Phase)  Ctag=CONS6  Atag=Signal  Itag=Irrad  Ttag=T_Amb  Wtag=Wind  HHtag=PQ_HH84  HHtagv=global  PVtag=PQ_PV84  PVtagv=global  EStag=PQ_ES84  EStagv=global  HPtag=PQ_HP84  HPtagv=global
      link override ES: Cap=32000  SoCin=0.7  Pin=15300  Pout=-15300
      link override HP: P_HP=4200  C=4590  H=241
      settings: SourceProductName=KIF2 Library
  HH85 : kif2/Household  Ctag=CONS7  Atag=Signal  Itag=Irrad  Ttag=T_Amb  Wtag=Wind  HHtag=PQ_HH85  HHtagv=global  PVtag=PQ_PV85  PVtagv=global  EStag=PQ_ES85  EStagv=global  HPtag=PQ_HP85  HPtagv=global
      link override ES: Cap=36500  SoCin=0.8  Pin=17300  Pout=-17300
      link override HP: P_HP=4800  C=5220  H=284
      link override PV: P_STCm=3100
      settings: SourceProductName=KIF2 Library
  HH86 : kif2/Household (Single Phase)  Ctag=CONS1  Atag=Signal  Itag=Irrad  Ttag=T_Amb  Wtag=Wind  HHtag=PQ_HH86  HHtagv=global  PVtag=PQ_PV86  PVtagv=global  EStag=PQ_ES86  EStagv=global  HPtag=PQ_HP86  HPtagv=global
      link override ES: Cap=9100  SoCin=0.2  Pin=5300  Pout=-5300
      link override HP: P_HP=2400  C=2655  H=140
      link override PV: P_STCm=800
      settings: SourceProductName=KIF2 Library
  HH87 : kif2/Household (Single Phase)  Ctag=CONS2  Atag=Signal  Itag=Irrad  Ttag=T_Amb  Wtag=Wind  HHtag=PQ_HH87  HHtagv=global  PVtag=PQ_PV87  PVtagv=global  EStag=PQ_ES87  EStagv=global  HPtag=PQ_HP87  HPtagv=global
      link override ES: Cap=13700  SoCin=0.3  Pin=7300  Pout=-7300
      link override HP: P_HP=3000  C=4950  H=141
      link override PV: P_STCm=1200
      settings: SourceProductName=KIF2 Library
  HH88 : kif2/Household (Single Phase)  Ctag=CONS3  Atag=Signal  Itag=Irrad  Ttag=T_Amb  Wtag=Wind  HHtag=PQ_HH88  HHtagv=global  PVtag=PQ_PV88  PVtagv=global  EStag=PQ_ES88  EStagv=global  HPtag=PQ_HP88  HPtagv=global
      link override ES: Cap=18300  SoCin=0.4  Pin=9300  Pout=-9300
      link override HP: P_HP=2500  C=2520  H=146
      link override PV: P_STCm=1500
      settings: SourceProductName=KIF2 Library
  HH89 : kif2/Household (Single Phase)  Ctag=CONS4  Atag=Signal  Itag=Irrad  Ttag=T_Amb  Wtag=Wind  HHtag=PQ_HH89  HHtagv=global  PVtag=PQ_PV89  PVtagv=global  EStag=PQ_ES89  EStagv=global  HPtag=PQ_HP89  HPtagv=global
      link override ES: Cap=22800  Pin=11300  Pout=-11300
      link override HP: P_HP=3300  C=4635  H=176
      link override PV: P_STCm=1900
      settings: SourceProductName=KIF2 Library
  HH9 : kif2/Household (Single Phase)  Ctag=CONS1  Atag=Signal  Itag=Irrad  Ttag=T_Amb  Wtag=Wind  HHtag=PQ_HH9  HHtagv=global  PVtag=PQ_PV9  PVtagv=global  EStag=PQ_ES9  EStagv=global  HPtag=PQ_HP9  HPtagv=global
      link override ES: Cap=9100  SoCin=0.2  Pin=5300  Pout=-5300
      link override HP: P_HP=2400  C=2655  H=140
      link override PV: P_STCm=800
      settings: SourceProductName=KIF2 Library
  HH90 : kif2/Household (Single Phase)  Ctag=CONS5  Atag=Signal  Itag=Irrad  Ttag=T_Amb  Wtag=Wind  HHtag=PQ_HH90  HHtagv=global  PVtag=PQ_PV90  PVtagv=global  EStag=PQ_ES90  EStagv=global  HPtag=PQ_HP90  HPtagv=global
      link override ES: Cap=27400  SoCin=0.6  Pin=13300  Pout=-13300
      link override PV: P_STCm=2300
      settings: SourceProductName=KIF2 Library
  HH91 : kif2/Household (Single Phase)  Ctag=CONS6  Atag=Signal  Itag=Irrad  Ttag=T_Amb  Wtag=Wind  HHtag=PQ_HH91  HHtagv=global  PVtag=PQ_PV91  PVtagv=global  EStag=PQ_ES91  EStagv=global  HPtag=PQ_HP91  HPtagv=global
      link override ES: Cap=32000  SoCin=0.7  Pin=15300  Pout=-15300
      link override HP: P_HP=4200  C=4590  H=241
      settings: SourceProductName=KIF2 Library
  HH92 : kif2/Household  Ctag=CONS7  Atag=Signal  Itag=Irrad  Ttag=T_Amb  Wtag=Wind  HHtag=PQ_HH92  HHtagv=global  PVtag=PQ_PV92  PVtagv=global  EStag=PQ_ES92  EStagv=global  HPtag=PQ_HP92  HPtagv=global
      link override ES: Cap=36500  SoCin=0.8  Pin=17300  Pout=-17300
      link override HP: P_HP=4800  C=5220  H=284
      link override PV: P_STCm=3100
      settings: SourceProductName=KIF2 Library
  HH93 : kif2/Household (Single Phase)  Ctag=CONS1  Atag=Signal  Itag=Irrad  Ttag=T_Amb  Wtag=Wind  HHtag=PQ_HH93  HHtagv=global  PVtag=PQ_PV93  PVtagv=global  EStag=PQ_ES93  EStagv=global  HPtag=PQ_HP93  HPtagv=global
      link override ES: Cap=9100  SoCin=0.2  Pin=5300  Pout=-5300
      link override HP: P_HP=2400  C=2655  H=140
      link override PV: P_STCm=800
      settings: SourceProductName=KIF2 Library
  HH94 : kif2/Household (Single Phase)  Ctag=CONS2  Atag=Signal  Itag=Irrad  Ttag=T_Amb  Wtag=Wind  HHtag=PQ_HH94  HHtagv=global  PVtag=PQ_PV94  PVtagv=global  EStag=PQ_ES94  EStagv=global  HPtag=PQ_HP94  HPtagv=global
      link override ES: Cap=13700  SoCin=0.3  Pin=7300  Pout=-7300
      link override HP: P_HP=3000  C=4950  H=141
      link override PV: P_STCm=1200
      settings: SourceProductName=KIF2 Library
  HH95 : kif2/Household (Single Phase)  Ctag=CONS3  Atag=Signal  Itag=Irrad  Ttag=T_Amb  Wtag=Wind  HHtag=PQ_HH95  HHtagv=global  PVtag=PQ_PV95  PVtagv=global  EStag=PQ_ES95  EStagv=global  HPtag=PQ_HP95  HPtagv=global
      link override ES: Cap=18300  SoCin=0.4  Pin=9300  Pout=-9300
      link override HP: P_HP=2500  C=2520  H=146
      link override PV: P_STCm=1500
      settings: SourceProductName=KIF2 Library
  HH96 : kif2/Household (Single Phase)  Ctag=CONS4  Atag=Signal  Itag=Irrad  Ttag=T_Amb  Wtag=Wind  HHtag=PQ_HH96  HHtagv=global  PVtag=PQ_PV96  PVtagv=global  EStag=PQ_ES96  EStagv=global  HPtag=PQ_HP96  HPtagv=global
      link override ES: Cap=22800  Pin=11300  Pout=-11300
      link override HP: P_HP=3300  C=4635  H=176
      link override PV: P_STCm=1900
      settings: SourceProductName=KIF2 Library
  HH97 : kif2/Household (Single Phase)  Ctag=CONS5  Atag=Signal  Itag=Irrad  Ttag=T_Amb  Wtag=Wind  HHtag=PQ_HH97  HHtagv=global  PVtag=PQ_PV97  PVtagv=global  EStag=PQ_ES97  EStagv=global  HPtag=PQ_HP97  HPtagv=global
      link override ES: Cap=27400  SoCin=0.6  Pin=13300  Pout=-13300
      link override PV: P_STCm=2300
      settings: SourceProductName=KIF2 Library
  HH98 : kif2/Household (Single Phase)  Ctag=CONS6  Atag=Signal  Itag=Irrad  Ttag=T_Amb  Wtag=Wind  HHtag=PQ_HH98  HHtagv=global  PVtag=PQ_PV98  PVtagv=global  EStag=PQ_ES98  EStagv=global  HPtag=PQ_HP98  HPtagv=global
      link override ES: Cap=32000  SoCin=0.7  Pin=15300  Pout=-15300
      link override HP: P_HP=4200  C=4590  H=241
      settings: SourceProductName=KIF2 Library
  HH99 : kif2/Household  Ctag=CONS7  Atag=Signal  Itag=Irrad  Ttag=T_Amb  Wtag=Wind  HHtag=PQ_HH99  HHtagv=global  PVtag=PQ_PV99  PVtagv=global  EStag=PQ_ES99  EStagv=global  HPtag=PQ_HP99  HPtagv=global
      link override ES: Cap=36500  SoCin=0.8  Pin=17300  Pout=-17300
      link override HP: P_HP=4800  C=5220  H=284
      link override PV: P_STCm=3100
      settings: SourceProductName=KIF2 Library
  Wire1 : kif2/Wire  Length=0.03  Frequency=50  Resistances=[296.8421e-003 446.8421e-003]  Inductances=[953.5880e-006 5.4671e-003]  Capacitances=[12.4583e-009 3.9055e-009]  Vtag=V_L1  Vtagv=global  Itag=I_L1  Itagv=global
      settings: SourceProductName=KIF2 Library
  Wire10 : kif2/Wire  Length=0.03  Frequency=50  Resistances=[296.8421e-003 446.8421e-003]  Inductances=[953.5880e-006 5.4671e-003]  Capacitances=[12.4583e-009 3.9055e-009]  Vtag=V_L10  Vtagv=global  Itag=I_L10  Itagv=global
      settings: SourceProductName=KIF2 Library
  Wire11 : kif2/Wire  Length=0.03  Frequency=50  Resistances=[296.8421e-003 446.8421e-003]  Inductances=[953.5880e-006 5.4671e-003]  Capacitances=[12.4583e-009 3.9055e-009]  Vtag=V_L11  Vtagv=global  Itag=I_L11  Itagv=global
      settings: SourceProductName=KIF2 Library
  Wire12 : kif2/Wire  Length=0.03  Frequency=50  Resistances=[296.8421e-003 446.8421e-003]  Inductances=[953.5880e-006 5.4671e-003]  Capacitances=[12.4583e-009 3.9055e-009]  Vtag=V_L12  Vtagv=global  Itag=I_L12  Itagv=global
      settings: SourceProductName=KIF2 Library
  Wire13 : kif2/Wire  Length=0.03  Frequency=50  Resistances=[296.8421e-003 446.8421e-003]  Inductances=[953.5880e-006 5.4671e-003]  Capacitances=[12.4583e-009 3.9055e-009]  Vtag=V_L13  Vtagv=global  Itag=I_L13  Itagv=global
      settings: SourceProductName=KIF2 Library
  Wire14 : kif2/Wire  Length=0.03  Frequency=50  Resistances=[564.0000e-003 714.0000e-003]  Inductances=[1.0178e-003 5.5313e-003]  Capacitances=[11.6151e-009 3.8190e-009]  Vtag=V_L14  Vtagv=global  Itag=I_L14  Itagv=global
      settings: SourceProductName=KIF2 Library
  Wire15 : kif2/Wire  Length=0.03  Frequency=50  Resistances=[296.8421e-003 446.8421e-003]  Inductances=[953.5880e-006 5.4671e-003]  Capacitances=[12.4583e-009 3.9055e-009]  Vtag=V_L15  Vtagv=global  Itag=I_L15  Itagv=global
      settings: SourceProductName=KIF2 Library
  Wire16 : kif2/Wire  Length=0.03  Frequency=50  Resistances=[296.8421e-003 446.8421e-003]  Inductances=[953.5880e-006 5.4671e-003]  Capacitances=[12.4583e-009 3.9055e-009]  Vtag=V_L16  Vtagv=global  Itag=I_L16  Itagv=global
      settings: SourceProductName=KIF2 Library
  Wire17 : kif2/Wire  Length=0.03  Frequency=50  Resistances=[296.8421e-003 446.8421e-003]  Inductances=[953.5880e-006 5.4671e-003]  Capacitances=[12.4583e-009 3.9055e-009]  Vtag=V_L17  Vtagv=global  Itag=I_L17  Itagv=global
      settings: SourceProductName=KIF2 Library
  Wire18 : kif2/Wire  Length=0.03  Frequency=50  Resistances=[296.8421e-003 446.8421e-003]  Inductances=[953.5880e-006 5.4671e-003]  Capacitances=[12.4583e-009 3.9055e-009]  Vtag=V_L18  Vtagv=global  Itag=I_L18  Itagv=global
      settings: SourceProductName=KIF2 Library
  Wire19 : kif2/Wire  Length=0.03  Frequency=50  Resistances=[296.8421e-003 446.8421e-003]  Inductances=[953.5880e-006 5.4671e-003]  Capacitances=[12.4583e-009 3.9055e-009]  Vtag=V_L19  Vtagv=global  Itag=I_L19  Itagv=global
      settings: SourceProductName=KIF2 Library
  Wire2 : kif2/Wire  Length=0.03  Frequency=50  Resistances=[296.8421e-003 446.8421e-003]  Inductances=[263.6030e-006 6.8471e-003]  Capacitances=[52.0885e-009 2.6280e-009]  Vtag=V_L2  Vtagv=global  Itag=I_L2  Itagv=global
      settings: SourceProductName=KIF2 Library
  Wire20 : kif2/Wire  Length=0.03  Frequency=50  Resistances=[296.8421e-003 446.8421e-003]  Inductances=[953.5880e-006 5.4671e-003]  Capacitances=[12.4583e-009 3.9055e-009]  Vtag=V_L20  Vtagv=global  Itag=I_L20  Itagv=global
      settings: SourceProductName=KIF2 Library
  Wire21 : kif2/Wire  Length=0.03  Frequency=50  Resistances=[296.8421e-003 446.8421e-003]  Inductances=[953.5880e-006 5.4671e-003]  Capacitances=[12.4583e-009 3.9055e-009]  Vtag=V_L21  Vtagv=global  Itag=I_L21  Itagv=global
      settings: SourceProductName=KIF2 Library
  Wire22 : kif2/Wire  Length=0.03  Frequency=50  Resistances=[564.0000e-003 714.0000e-003]  Inductances=[1.0178e-003 5.5313e-003]  Capacitances=[11.6151e-009 3.8190e-009]  Vtag=V_L22  Vtagv=global  Itag=I_L22  Itagv=global
      settings: SourceProductName=KIF2 Library
  Wire23 : kif2/Wire  Length=0.03  Frequency=50  Resistances=[296.8421e-003 446.8421e-003]  Inductances=[953.5880e-006 5.4671e-003]  Capacitances=[12.4583e-009 3.9055e-009]  Vtag=V_L23  Vtagv=global  Itag=I_L23  Itagv=global
      settings: SourceProductName=KIF2 Library
  Wire24 : kif2/Wire  Length=0.03  Frequency=50  Resistances=[296.8421e-003 446.8421e-003]  Inductances=[953.5880e-006 5.4671e-003]  Capacitances=[12.4583e-009 3.9055e-009]  Vtag=V_L24  Vtagv=global  Itag=I_L24  Itagv=global
      settings: SourceProductName=KIF2 Library
  Wire25 : kif2/Wire  Length=0.03  Frequency=50  Resistances=[296.8421e-003 446.8421e-003]  Inductances=[953.5880e-006 5.4671e-003]  Capacitances=[12.4583e-009 3.9055e-009]  Vtag=V_L25  Vtagv=global  Itag=I_L25  Itagv=global
      settings: SourceProductName=KIF2 Library
  Wire26 : kif2/Wire  Length=0.03  Frequency=50  Resistances=[564.0000e-003 714.0000e-003]  Inductances=[1.0178e-003 5.5313e-003]  Capacitances=[11.6151e-009 3.8190e-009]  Vtag=V_L26  Vtagv=global  Itag=I_L26  Itagv=global
      settings: SourceProductName=KIF2 Library
  Wire27 : kif2/Wire  Length=0.03  Frequency=50  Resistances=[296.8421e-003 446.8421e-003]  Inductances=[953.5880e-006 5.4671e-003]  Capacitances=[12.4583e-009 3.9055e-009]  Vtag=V_L27  Vtagv=global  Itag=I_L27  Itagv=global
      settings: SourceProductName=KIF2 Library
  Wire28 : kif2/Wire  Length=0.03  Frequency=50  Resistances=[296.8421e-003 446.8421e-003]  Inductances=[953.5880e-006 5.4671e-003]  Capacitances=[12.4583e-009 3.9055e-009]  Vtag=V_L28  Vtagv=global  Itag=I_L28  Itagv=global
      settings: SourceProductName=KIF2 Library
  Wire29 : kif2/Wire  Length=0.03  Frequency=50  Resistances=[296.8421e-003 446.8421e-003]  Inductances=[953.5880e-006 5.4671e-003]  Capacitances=[12.4583e-009 3.9055e-009]  Vtag=V_L29  Vtagv=global  Itag=I_L29  Itagv=global
      settings: SourceProductName=KIF2 Library
  Wire3 : kif2/Wire  Length=0.03  Frequency=50  Resistances=[188.0000e-003 338.0000e-003]  Inductances=[630.6533e-006 5.9760e-003]  Capacitances=[872.4959e-009 872.4959e-009]  Vtag=V_L3  Vtagv=global  Itag=I_L3  Itagv=global
      settings: SourceProductName=KIF2 Library
  Wire30 : kif2/Wire  Length=0.03  Frequency=50  Resistances=[296.8421e-003 446.8421e-003]  Inductances=[953.5880e-006 5.4671e-003]  Capacitances=[12.4583e-009 3.9055e-009]  Vtag=V_L30  Vtagv=global  Itag=I_L30  Itagv=global
      settings: SourceProductName=KIF2 Library
  Wire31 : kif2/Wire  Length=0.03  Frequency=50  Resistances=[296.8421e-003 446.8421e-003]  Inductances=[953.5880e-006 5.4671e-003]  Capacitances=[12.4583e-009 3.9055e-009]  Vtag=V_L31  Vtagv=global  Itag=I_L31  Itagv=global
      settings: SourceProductName=KIF2 Library
  Wire32 : kif2/Wire  Length=0.03  Frequency=50  Resistances=[564.0000e-003 714.0000e-003]  Inductances=[1.0178e-003 5.5313e-003]  Capacitances=[11.6151e-009 3.8190e-009]  Vtag=V_L32  Vtagv=global  Itag=I_L32  Itagv=global
      settings: SourceProductName=KIF2 Library
  Wire33 : kif2/Wire  Length=0.03  Frequency=50  Resistances=[564.0000e-003 714.0000e-003]  Inductances=[1.0178e-003 5.5313e-003]  Capacitances=[11.6151e-009 3.8190e-009]  Vtag=V_L33  Vtagv=global  Itag=I_L33  Itagv=global
      settings: SourceProductName=KIF2 Library
  Wire34 : kif2/Wire  Length=0.03  Frequency=50  Resistances=[564.0000e-003 714.0000e-003]  Inductances=[1.0178e-003 5.5313e-003]  Capacitances=[11.6151e-009 3.8190e-009]  Vtag=V_L34  Vtagv=global  Itag=I_L34  Itagv=global
      settings: SourceProductName=KIF2 Library
  Wire35 : kif2/Wire  Length=0.03  Frequency=50  Resistances=[564.0000e-003 714.0000e-003]  Inductances=[1.0178e-003 5.5313e-003]  Capacitances=[11.6151e-009 3.8190e-009]  Vtag=V_L35  Vtagv=global  Itag=I_L35  Itagv=global
      settings: SourceProductName=KIF2 Library
  Wire36 : kif2/Wire  Length=0.03  Frequency=50  Resistances=[564.0000e-003 714.0000e-003]  Inductances=[1.0178e-003 5.5313e-003]  Capacitances=[11.6151e-009 3.8190e-009]  Vtag=V_L36  Vtagv=global  Itag=I_L36  Itagv=global
      settings: SourceProductName=KIF2 Library
  Wire37 : kif2/Wire  Length=0.03  Frequency=50  Resistances=[564.0000e-003 714.0000e-003]  Inductances=[1.0178e-003 5.5313e-003]  Capacitances=[11.6151e-009 3.8190e-009]  Vtag=V_L37  Vtagv=global  Itag=I_L37  Itagv=global
      settings: SourceProductName=KIF2 Library
  Wire38 : kif2/Wire  Length=0.03  Frequency=50  Resistances=[564.0000e-003 714.0000e-003]  Inductances=[1.0178e-003 5.5313e-003]  Capacitances=[11.6151e-009 3.8190e-009]  Vtag=V_L38  Vtagv=global  Itag=I_L38  Itagv=global
      settings: SourceProductName=KIF2 Library
  Wire39 : kif2/Wire  Length=0.03  Frequency=50  Resistances=[564.0000e-003 714.0000e-003]  Inductances=[1.0178e-003 5.5313e-003]  Capacitances=[11.6151e-009 3.8190e-009]  Vtag=V_L39  Vtagv=global  Itag=I_L39  Itagv=global
      settings: SourceProductName=KIF2 Library
  Wire4 : kif2/Wire  Length=0.03  Frequency=50  Resistances=[296.8421e-003 446.8421e-003]  Inductances=[953.5880e-006 5.4671e-003]  Capacitances=[12.4583e-009 3.9055e-009]  Vtag=V_L4  Vtagv=global  Itag=I_L4  Itagv=global
      settings: SourceProductName=KIF2 Library
  Wire40 : kif2/Wire  Length=0.03  Frequency=50  Resistances=[564.0000e-003 714.0000e-003]  Inductances=[1.0178e-003 5.5313e-003]  Capacitances=[11.6151e-009 3.8190e-009]  Vtag=V_L40  Vtagv=global  Itag=I_L40  Itagv=global
      settings: SourceProductName=KIF2 Library
  Wire41 : kif2/Wire  Length=0.03  Frequency=50  Resistances=[564.0000e-003 714.0000e-003]  Inductances=[1.0178e-003 5.5313e-003]  Capacitances=[11.6151e-009 3.8190e-009]  Vtag=V_L41  Vtagv=global  Itag=I_L41  Itagv=global
      settings: SourceProductName=KIF2 Library
  Wire42 : kif2/Wire  Length=0.03  Frequency=50  Resistances=[564.0000e-003 714.0000e-003]  Inductances=[1.0178e-003 5.5313e-003]  Capacitances=[11.6151e-009 3.8190e-009]  Vtag=V_L42  Vtagv=global  Itag=I_L42  Itagv=global
      settings: SourceProductName=KIF2 Library
  Wire43 : kif2/Wire  Length=0.03  Frequency=50  Resistances=[564.0000e-003 714.0000e-003]  Inductances=[1.0178e-003 5.5313e-003]  Capacitances=[11.6151e-009 3.8190e-009]  Vtag=V_L43  Vtagv=global  Itag=I_L43  Itagv=global
      settings: SourceProductName=KIF2 Library
  Wire44 : kif2/Wire  Length=0.03  Frequency=50  Resistances=[564.0000e-003 714.0000e-003]  Inductances=[1.0178e-003 5.5313e-003]  Capacitances=[11.6151e-009 3.8190e-009]  Vtag=V_L44  Vtagv=global  Itag=I_L44  Itagv=global
      settings: SourceProductName=KIF2 Library
  Wire45 : kif2/Wire  Length=0.03  Frequency=50  Resistances=[564.0000e-003 714.0000e-003]  Inductances=[1.0178e-003 5.5313e-003]  Capacitances=[11.6151e-009 3.8190e-009]  Vtag=V_L45  Vtagv=global  Itag=I_L45  Itagv=global
      settings: SourceProductName=KIF2 Library
  Wire46 : kif2/Wire  Length=0.03  Frequency=50  Resistances=[564.0000e-003 714.0000e-003]  Inductances=[1.0178e-003 5.5313e-003]  Capacitances=[11.6151e-009 3.8190e-009]  Vtag=V_L46  Vtagv=global  Itag=I_L46  Itagv=global
      settings: SourceProductName=KIF2 Library
  Wire47 : kif2/Wire  Length=0.03  Frequency=50  Resistances=[564.0000e-003 714.0000e-003]  Inductances=[1.0178e-003 5.5313e-003]  Capacitances=[11.6151e-009 3.8190e-009]  Vtag=V_L47  Vtagv=global  Itag=I_L47  Itagv=global
      settings: SourceProductName=KIF2 Library
  Wire48 : kif2/Wire  Length=0.03  Frequency=50  Resistances=[564.0000e-003 714.0000e-003]  Inductances=[1.0178e-003 5.5313e-003]  Capacitances=[11.6151e-009 3.8190e-009]  Vtag=V_L48  Vtagv=global  Itag=I_L48  Itagv=global
      settings: SourceProductName=KIF2 Library
  Wire49 : kif2/Wire  Length=0.03  Frequency=50  Resistances=[564.0000e-003 714.0000e-003]  Inductances=[1.0178e-003 5.5313e-003]  Capacitances=[11.6151e-009 3.8190e-009]  Vtag=V_L49  Vtagv=global  Itag=I_L49  Itagv=global
      settings: SourceProductName=KIF2 Library
  Wire5 : kif2/Wire  Length=0.03  Frequency=50  Resistances=[296.8421e-003 446.8421e-003]  Inductances=[953.5880e-006 5.4671e-003]  Capacitances=[12.4583e-009 3.9055e-009]  Vtag=V_L5  Vtagv=global  Itag=I_L5  Itagv=global
      settings: SourceProductName=KIF2 Library
  Wire50 : kif2/Wire  Length=0.03  Frequency=50  Resistances=[564.0000e-003 714.0000e-003]  Inductances=[1.0178e-003 5.5313e-003]  Capacitances=[11.6151e-009 3.8190e-009]  Vtag=V_L50  Vtagv=global  Itag=I_L50  Itagv=global
      settings: SourceProductName=KIF2 Library
  Wire51 : kif2/Wire  Length=0.03  Frequency=50  Resistances=[564.0000e-003 714.0000e-003]  Inductances=[1.0178e-003 5.5313e-003]  Capacitances=[11.6151e-009 3.8190e-009]  Vtag=V_L51  Vtagv=global  Itag=I_L51  Itagv=global
      settings: SourceProductName=KIF2 Library
  Wire52 : kif2/Wire  Length=0.03  Frequency=50  Resistances=[564.0000e-003 714.0000e-003]  Inductances=[1.0178e-003 5.5313e-003]  Capacitances=[11.6151e-009 3.8190e-009]  Vtag=V_L52  Vtagv=global  Itag=I_L52  Itagv=global
      settings: SourceProductName=KIF2 Library
  Wire53 : kif2/Wire  Length=0.03  Frequency=50  Resistances=[564.0000e-003 714.0000e-003]  Inductances=[1.0178e-003 5.5313e-003]  Capacitances=[11.6151e-009 3.8190e-009]  Vtag=V_L53  Vtagv=global  Itag=I_L53  Itagv=global
      settings: SourceProductName=KIF2 Library
  Wire54 : kif2/Wire  Length=0.03  Frequency=50  Resistances=[296.8421e-003 446.8421e-003]  Inductances=[263.6030e-006 6.8471e-003]  Capacitances=[52.0885e-009 2.6280e-009]  Vtag=V_L54  Vtagv=global  Itag=I_L54  Itagv=global
      settings: SourceProductName=KIF2 Library
  Wire55 : kif2/Wire  Length=0.03  Frequency=50  Resistances=[296.8421e-003 446.8421e-003]  Inductances=[263.6030e-006 6.8471e-003]  Capacitances=[52.0885e-009 2.6280e-009]  Vtag=V_L55  Vtagv=global  Itag=I_L55  Itagv=global
      settings: SourceProductName=KIF2 Library
  Wire56 : kif2/Wire  Length=0.03  Frequency=50  Resistances=[296.8421e-003 446.8421e-003]  Inductances=[263.6030e-006 6.8471e-003]  Capacitances=[52.0885e-009 2.6280e-009]  Vtag=V_L56  Vtagv=global  Itag=I_L56  Itagv=global
      settings: SourceProductName=KIF2 Library
  Wire57 : kif2/Wire  Length=0.03  Frequency=50  Resistances=[296.8421e-003 446.8421e-003]  Inductances=[263.6030e-006 6.8471e-003]  Capacitances=[52.0885e-009 2.6280e-009]  Vtag=V_L57  Vtagv=global  Itag=I_L57  Itagv=global
      settings: SourceProductName=KIF2 Library
  Wire58 : kif2/Wire  Length=0.03  Frequency=50  Resistances=[296.8421e-003 446.8421e-003]  Inductances=[263.6030e-006 6.8471e-003]  Capacitances=[52.0885e-009 2.6280e-009]  Vtag=V_L58  Vtagv=global  Itag=I_L58  Itagv=global
      settings: SourceProductName=KIF2 Library
  Wire59 : kif2/Wire  Length=0.03  Frequency=50  Resistances=[296.8421e-003 446.8421e-003]  Inductances=[263.6030e-006 6.8471e-003]  Capacitances=[52.0885e-009 2.6280e-009]  Vtag=V_L59  Vtagv=global  Itag=I_L59  Itagv=global
      settings: SourceProductName=KIF2 Library
  Wire6 : kif2/Wire  Length=0.03  Frequency=50  Resistances=[296.8421e-003 446.8421e-003]  Inductances=[953.5880e-006 5.4671e-003]  Capacitances=[12.4583e-009 3.9055e-009]  Vtag=V_L6  Vtagv=global  Itag=I_L6  Itagv=global
      settings: SourceProductName=KIF2 Library
  Wire60 : kif2/Wire  Length=0.03  Frequency=50  Resistances=[296.8421e-003 446.8421e-003]  Inductances=[263.6030e-006 6.8471e-003]  Capacitances=[52.0885e-009 2.6280e-009]  Vtag=V_L60  Vtagv=global  Itag=I_L60  Itagv=global
      settings: SourceProductName=KIF2 Library
  Wire61 : kif2/Wire  Length=0.03  Frequency=50  Resistances=[296.8421e-003 446.8421e-003]  Inductances=[263.6030e-006 6.8471e-003]  Capacitances=[52.0885e-009 2.6280e-009]  Vtag=V_L61  Vtagv=global  Itag=I_L61  Itagv=global
      settings: SourceProductName=KIF2 Library
  Wire62 : kif2/Wire  Length=0.03  Frequency=50  Resistances=[263.6030e-006 6.8471e-003]  Inductances=[270.2520e-006 7.0263e-003]  Capacitances=[50.5161e-009 2.5213e-009]  Vtag=V_L62  Vtagv=global  Itag=I_L62  Itagv=global
      settings: SourceProductName=KIF2 Library
  Wire63 : kif2/Wire  Length=0.03  Frequency=50  Resistances=[296.8421e-003 446.8421e-003]  Inductances=[263.6030e-006 6.8471e-003]  Capacitances=[52.0885e-009 2.6280e-009]  Vtag=V_L63  Vtagv=global  Itag=I_L63  Itagv=global
      settings: SourceProductName=KIF2 Library
  Wire64 : kif2/Wire  Length=0.03  Frequency=50  Resistances=[296.8421e-003 446.8421e-003]  Inductances=[263.6030e-006 6.8471e-003]  Capacitances=[52.0885e-009 2.6280e-009]  Vtag=V_L64  Vtagv=global  Itag=I_L64  Itagv=global
      settings: SourceProductName=KIF2 Library
  Wire65 : kif2/Wire  Length=0.03  Frequency=50  Resistances=[296.8421e-003 446.8421e-003]  Inductances=[263.6030e-006 6.8471e-003]  Capacitances=[52.0885e-009 2.6280e-009]  Vtag=V_L65  Vtagv=global  Itag=I_L65  Itagv=global
      settings: SourceProductName=KIF2 Library
  Wire66 : kif2/Wire  Length=0.03  Frequency=50  Resistances=[296.8421e-003 446.8421e-003]  Inductances=[263.6030e-006 6.8471e-003]  Capacitances=[52.0885e-009 2.6280e-009]  Vtag=V_L66  Vtagv=global  Itag=I_L66  Itagv=global
      settings: SourceProductName=KIF2 Library
  Wire67 : kif2/Wire  Length=0.03  Frequency=50  Resistances=[296.8421e-003 446.8421e-003]  Inductances=[263.6030e-006 6.8471e-003]  Capacitances=[52.0885e-009 2.6280e-009]  Vtag=V_L67  Vtagv=global  Itag=I_L67  Itagv=global
      settings: SourceProductName=KIF2 Library
  Wire68 : kif2/Wire  Length=0.03  Frequency=50  Resistances=[296.8421e-003 446.8421e-003]  Inductances=[263.6030e-006 6.8471e-003]  Capacitances=[52.0885e-009 2.6280e-009]  Vtag=V_L68  Vtagv=global  Itag=I_L68  Itagv=global
      settings: SourceProductName=KIF2 Library
  Wire69 : kif2/Wire  Length=0.03  Frequency=50  Resistances=[263.6030e-006 6.8471e-003]  Inductances=[270.2520e-006 7.0263e-003]  Capacitances=[50.5161e-009 2.5213e-009]  Vtag=V_L69  Vtagv=global  Itag=I_L69  Itagv=global
      settings: SourceProductName=KIF2 Library
  Wire7 : kif2/Wire  Length=0.03  Frequency=50  Resistances=[296.8421e-003 446.8421e-003]  Inductances=[953.5880e-006 5.4671e-003]  Capacitances=[12.4583e-009 3.9055e-009]  Vtag=V_L7  Vtagv=global  Itag=I_L7  Itagv=global
      settings: SourceProductName=KIF2 Library
  Wire70 : kif2/Wire  Length=0.03  Frequency=50  Resistances=[263.6030e-006 6.8471e-003]  Inductances=[270.2520e-006 7.0263e-003]  Capacitances=[50.5161e-009 2.5213e-009]  Vtag=V_L70  Vtagv=global  Itag=I_L70  Itagv=global
      settings: SourceProductName=KIF2 Library
  Wire71 : kif2/Wire  Length=0.03  Frequency=50  Resistances=[263.6030e-006 6.8471e-003]  Inductances=[270.2520e-006 7.0263e-003]  Capacitances=[50.5161e-009 2.5213e-009]  Vtag=V_L71  Vtagv=global  Itag=I_L71  Itagv=global
      settings: SourceProductName=KIF2 Library
  Wire72 : kif2/Wire  Length=0.03  Frequency=50  Resistances=[263.6030e-006 6.8471e-003]  Inductances=[270.2520e-006 7.0263e-003]  Capacitances=[50.5161e-009 2.5213e-009]  Vtag=V_L72  Vtagv=global  Itag=I_L72  Itagv=global
      settings: SourceProductName=KIF2 Library
  Wire73 : kif2/Wire  Length=0.03  Frequency=50  Resistances=[263.6030e-006 6.8471e-003]  Inductances=[270.2520e-006 7.0263e-003]  Capacitances=[50.5161e-009 2.5213e-009]  Vtag=V_L73  Vtagv=global  Itag=I_L73  Itagv=global
      settings: SourceProductName=KIF2 Library
  Wire74 : kif2/Wire  Length=0.03  Frequency=50  Resistances=[263.6030e-006 6.8471e-003]  Inductances=[270.2520e-006 7.0263e-003]  Capacitances=[50.5161e-009 2.5213e-009]  Vtag=V_L74  Vtagv=global  Itag=I_L74  Itagv=global
      settings: SourceProductName=KIF2 Library
  Wire75 : kif2/Wire  Length=0.03  Frequency=50  Resistances=[188.0000e-003 338.0000e-003]  Inductances=[630.6533e-006 5.9760e-003]  Capacitances=[872.4959e-009 872.4959e-009]  Vtag=V_L75  Vtagv=global  Itag=I_L75  Itagv=global
      settings: SourceProductName=KIF2 Library
  Wire76 : kif2/Wire  Length=0.03  Frequency=50  Resistances=[188.0000e-003 338.0000e-003]  Inductances=[630.6533e-006 5.9760e-003]  Capacitances=[872.4959e-009 872.4959e-009]  Vtag=V_L76  Vtagv=global  Itag=I_L76  Itagv=global
      settings: SourceProductName=KIF2 Library
  Wire77 : kif2/Wire  Length=0.03  Frequency=50  Resistances=[188.0000e-003 338.0000e-003]  Inductances=[630.6533e-006 5.9760e-003]  Capacitances=[872.4959e-009 872.4959e-009]  Vtag=V_L77  Vtagv=global  Itag=I_L77  Itagv=global
      settings: SourceProductName=KIF2 Library
  Wire78 : kif2/Wire  Length=0.03  Frequency=50  Resistances=[188.0000e-003 338.0000e-003]  Inductances=[630.6533e-006 5.9760e-003]  Capacitances=[872.4959e-009 872.4959e-009]  Vtag=V_L78  Vtagv=global  Itag=I_L78  Itagv=global
      settings: SourceProductName=KIF2 Library
  Wire79 : kif2/Wire  Length=0.03  Frequency=50  Resistances=[188.0000e-003 338.0000e-003]  Inductances=[630.6533e-006 5.9760e-003]  Capacitances=[872.4959e-009 872.4959e-009]  Vtag=V_L79  Vtagv=global  Itag=I_L79  Itagv=global
      settings: SourceProductName=KIF2 Library
  Wire8 : kif2/Wire  Length=0.03  Frequency=50  Resistances=[296.8421e-003 446.8421e-003]  Inductances=[953.5880e-006 5.4671e-003]  Capacitances=[12.4583e-009 3.9055e-009]  Vtag=V_L8  Vtagv=global  Itag=I_L8  Itagv=global
      settings: SourceProductName=KIF2 Library
  Wire80 : kif2/Wire  Length=0.03  Frequency=50  Resistances=[188.0000e-003 338.0000e-003]  Inductances=[630.6533e-006 5.9760e-003]  Capacitances=[872.4959e-009 872.4959e-009]  Vtag=V_L80  Vtagv=global  Itag=I_L80  Itagv=global
      settings: SourceProductName=KIF2 Library
  Wire81 : kif2/Wire  Length=0.03  Frequency=50  Resistances=[188.0000e-003 338.0000e-003]  Inductances=[630.6533e-006 5.9760e-003]  Capacitances=[872.4959e-009 872.4959e-009]  Vtag=V_L81  Vtagv=global  Itag=I_L81  Itagv=global
      settings: SourceProductName=KIF2 Library
  Wire82 : kif2/Wire  Length=0.03  Frequency=50  Resistances=[188.0000e-003 338.0000e-003]  Inductances=[630.6533e-006 5.9760e-003]  Capacitances=[872.4959e-009 872.4959e-009]  Vtag=V_L82  Vtagv=global  Itag=I_L82  Itagv=global
      settings: SourceProductName=KIF2 Library
  Wire83 : kif2/Wire  Length=0.03  Frequency=50  Resistances=[188.0000e-003 338.0000e-003]  Inductances=[630.6533e-006 5.9760e-003]  Capacitances=[872.4959e-009 872.4959e-009]  Vtag=V_L83  Vtagv=global  Itag=I_L83  Itagv=global
      settings: SourceProductName=KIF2 Library
  Wire84 : kif2/Wire  Length=0.03  Frequency=50  Resistances=[188.0000e-003 338.0000e-003]  Inductances=[630.6533e-006 5.9760e-003]  Capacitances=[872.4959e-009 872.4959e-009]  Vtag=V_L84  Vtagv=global  Itag=I_L84  Itagv=global
      settings: SourceProductName=KIF2 Library
  Wire85 : kif2/Wire  Length=0.03  Frequency=50  Resistances=[188.0000e-003 338.0000e-003]  Inductances=[630.6533e-006 5.9760e-003]  Capacitances=[872.4959e-009 872.4959e-009]  Vtag=V_L85  Vtagv=global  Itag=I_L85  Itagv=global
      settings: SourceProductName=KIF2 Library
  Wire86 : kif2/Wire  Length=0.03  Frequency=50  Resistances=[188.0000e-003 338.0000e-003]  Inductances=[630.6533e-006 5.9760e-003]  Capacitances=[872.4959e-009 872.4959e-009]  Vtag=V_L86  Vtagv=global  Itag=I_L86  Itagv=global
      settings: SourceProductName=KIF2 Library
  Wire87 : kif2/Wire  Length=0.03  Frequency=50  Resistances=[188.0000e-003 338.0000e-003]  Inductances=[630.6533e-006 5.9760e-003]  Capacitances=[872.4959e-009 872.4959e-009]  Vtag=V_L87  Vtagv=global  Itag=I_L87  Itagv=global
      settings: SourceProductName=KIF2 Library
  Wire88 : kif2/Wire  Length=0.03  Frequency=50  Resistances=[188.0000e-003 338.0000e-003]  Inductances=[630.6533e-006 5.9760e-003]  Capacitances=[872.4959e-009 872.4959e-009]  Vtag=V_L88  Vtagv=global  Itag=I_L88  Itagv=global
      settings: SourceProductName=KIF2 Library
  Wire9 : kif2/Wire  Length=0.03  Frequency=50  Resistances=[296.8421e-003 446.8421e-003]  Inductances=[953.5880e-006 5.4671e-003]  Capacitances=[12.4583e-009 3.9055e-009]  Vtag=V_L9  Vtagv=global  Itag=I_L9  Itagv=global
      settings: SourceProductName=KIF2 Library
  connections:
  HH1/LConn1 -- Wire1/RConn1 -- Wire4/LConn1
  HH1/LConn2 -- Wire1/RConn2 -- Wire4/LConn2
  HH1/LConn3 -- Wire1/RConn3 -- Wire4/LConn3
  HH2/LConn1 -- Wire4/RConn1 -- Wire5/LConn1
  HH3/LConn1 -- Wire4/RConn2 -- Wire5/LConn2
  HH4/LConn1 -- Wire4/RConn3 -- Wire5/LConn3
  HH5/LConn1 -- Wire5/RConn1 -- Wire6/LConn1
  HH6/LConn1 -- Wire5/RConn2 -- Wire6/LConn2
  HH7/LConn1 -- Wire5/RConn3 -- Wire6/LConn3
  HH8/LConn1 -- Wire6/RConn1 -- Wire7/LConn1
  HH8/LConn2 -- Wire6/RConn2 -- Wire7/LConn2
  HH8/LConn3 -- Wire6/RConn3 -- Wire7/LConn3
  HH9/LConn1 -- Wire7/RConn1 -- Wire8/LConn1
  HH10/LConn1 -- Wire7/RConn2 -- Wire8/LConn2
  HH11/LConn1 -- Wire7/RConn3 -- Wire8/LConn3
  HH12/LConn1 -- Wire8/RConn1 -- Wire9/LConn1
  HH13/LConn1 -- Wire8/RConn2 -- Wire9/LConn2
  HH14/LConn1 -- Wire8/RConn3 -- Wire9/LConn3
  HH15/LConn1 -- Wire9/RConn1 -- Wire10/LConn1
  HH15/LConn2 -- Wire9/RConn2 -- Wire10/LConn2
  HH15/LConn3 -- Wire9/RConn3 -- Wire10/LConn3
  HH16/LConn1 -- Wire10/RConn1 -- Wire11/LConn1
  HH17/LConn1 -- Wire10/RConn2 -- Wire11/LConn2
  HH18/LConn1 -- Wire10/RConn3 -- Wire11/LConn3
  HH19/LConn1 -- Wire11/RConn1 -- Wire12/LConn1
  HH20/LConn1 -- Wire11/RConn2 -- Wire12/LConn2
  HH21/LConn1 -- Wire11/RConn3 -- Wire12/LConn3
  HH22/LConn1 -- Wire12/RConn1 -- Wire13/LConn1 -- Wire14/LConn1
  HH22/LConn2 -- Wire12/RConn2 -- Wire13/LConn2 -- Wire14/LConn2
  HH22/LConn3 -- Wire12/RConn3 -- Wire13/LConn3 -- Wire14/LConn3
  HH23/LConn1 -- Wire13/RConn1 -- Wire15/LConn1
  HH24/LConn1 -- Wire13/RConn2 -- Wire15/LConn2
  HH25/LConn1 -- Wire13/RConn3 -- Wire15/LConn3
  HH26/LConn1 -- Wire15/RConn1 -- Wire16/LConn1
  HH27/LConn1 -- Wire15/RConn2 -- Wire16/LConn2
  HH28/LConn1 -- Wire15/RConn3 -- Wire16/LConn3
  HH29/LConn1 -- Wire16/RConn1 -- Wire17/LConn1
  HH29/LConn2 -- Wire16/RConn2 -- Wire17/LConn2
  HH29/LConn3 -- Wire16/RConn3 -- Wire17/LConn3
  HH30/LConn1 -- Wire17/RConn1 -- Wire18/LConn1
  HH31/LConn1 -- Wire17/RConn2 -- Wire18/LConn2
  HH32/LConn1 -- Wire17/RConn3 -- Wire18/LConn3
  HH33/LConn1 -- Wire18/RConn1 -- Wire19/LConn1
  HH34/LConn1 -- Wire18/RConn2 -- Wire19/LConn2
  HH35/LConn1 -- Wire18/RConn3 -- Wire19/LConn3
  HH36/LConn1 -- Wire19/RConn1 -- Wire20/LConn1
  HH36/LConn2 -- Wire19/RConn2 -- Wire20/LConn2
  HH36/LConn3 -- Wire19/RConn3 -- Wire20/LConn3
  HH37/LConn1 -- Wire20/RConn1 -- Wire21/LConn1 -- Wire22/LConn1
  HH38/LConn1 -- Wire20/RConn2 -- Wire21/LConn2 -- Wire22/LConn2
  HH39/LConn1 -- Wire20/RConn3 -- Wire21/LConn3 -- Wire22/LConn3
  HH40/LConn1 -- Wire21/RConn1 -- Wire23/LConn1
  HH41/LConn1 -- Wire21/RConn2 -- Wire23/LConn2
  HH42/LConn1 -- Wire21/RConn3 -- Wire23/LConn3
  HH43/LConn1 -- Wire23/RConn1 -- Wire24/LConn1
  HH43/LConn2 -- Wire23/RConn2 -- Wire24/LConn2
  HH43/LConn3 -- Wire23/RConn3 -- Wire24/LConn3
  HH44/LConn1 -- Wire24/RConn1 -- Wire25/LConn1 -- Wire26/LConn1
  HH45/LConn1 -- Wire24/RConn2 -- Wire25/LConn2 -- Wire26/LConn2
  HH46/LConn1 -- Wire24/RConn3 -- Wire25/LConn3 -- Wire26/LConn3
  HH47/LConn1 -- Wire25/RConn1 -- Wire27/LConn1
  HH48/LConn1 -- Wire25/RConn2 -- Wire27/LConn2
  HH49/LConn1 -- Wire25/RConn3 -- Wire27/LConn3
  HH50/LConn1 -- Wire27/RConn1 -- Wire28/LConn1
  HH50/LConn2 -- Wire27/RConn2 -- Wire28/LConn2
  HH50/LConn3 -- Wire27/RConn3 -- Wire28/LConn3
  HH51/LConn1 -- Wire28/RConn1 -- Wire29/LConn1
  HH52/LConn1 -- Wire28/RConn2 -- Wire29/LConn2
  HH53/LConn1 -- Wire28/RConn3 -- Wire29/LConn3
  HH54/LConn1 -- Wire29/RConn1 -- Wire30/LConn1
  HH55/LConn1 -- Wire29/RConn2 -- Wire30/LConn2
  HH56/LConn1 -- Wire29/RConn3 -- Wire30/LConn3
  HH57/LConn1 -- Wire30/RConn1 -- Wire31/LConn1
  HH57/LConn2 -- Wire30/RConn2 -- Wire31/LConn2
  HH57/LConn3 -- Wire30/RConn3 -- Wire31/LConn3
  HH58/LConn1 -- Wire31/RConn1 -- Wire32/LConn1
  HH59/LConn1 -- Wire31/RConn2 -- Wire32/LConn2
  HH60/LConn1 -- Wire31/RConn3 -- Wire32/LConn3
  HH61/LConn1 -- Wire32/RConn1 -- Wire33/LConn1
  HH62/LConn1 -- Wire32/RConn2 -- Wire33/LConn2
  HH63/LConn1 -- Wire32/RConn3 -- Wire33/LConn3
  HH64/LConn1 -- Wire33/RConn1 -- Wire34/LConn1
  HH64/LConn2 -- Wire33/RConn2 -- Wire34/LConn2
  HH64/LConn3 -- Wire33/RConn3 -- Wire34/LConn3
  HH65/LConn1 -- Wire34/RConn1 -- Wire35/LConn1
  HH66/LConn1 -- Wire34/RConn2 -- Wire35/LConn2
  HH67/LConn1 -- Wire34/RConn3 -- Wire35/LConn3
  HH68/LConn1 -- Wire35/RConn1 -- Wire36/LConn1
  HH69/LConn1 -- Wire35/RConn2 -- Wire36/LConn2
  HH70/LConn1 -- Wire35/RConn3 -- Wire36/LConn3
  HH71/LConn1 -- Wire36/RConn1 -- Wire37/LConn1
  HH71/LConn2 -- Wire36/RConn2 -- Wire37/LConn2
  HH71/LConn3 -- Wire36/RConn3 -- Wire37/LConn3
  HH72/LConn1 -- Wire37/RConn1 -- Wire38/LConn1
  HH73/LConn1 -- Wire37/RConn2 -- Wire38/LConn2
  HH74/LConn1 -- Wire37/RConn3 -- Wire38/LConn3
  Wire38/RConn1 -- HH75/LConn1
  Wire38/RConn2 -- HH76/LConn1
  Wire38/RConn3 -- HH77/LConn1
  HH78/LConn1 -- Wire26/RConn1 -- Wire49/LConn1
  HH78/LConn2 -- Wire26/RConn2 -- Wire49/LConn2
  HH78/LConn3 -- Wire26/RConn3 -- Wire49/LConn3
  HH79/LConn1 -- Wire49/RConn1 -- Wire50/LConn1
  HH80/LConn1 -- Wire49/RConn2 -- Wire50/LConn2
  HH81/LConn1 -- Wire49/RConn3 -- Wire50/LConn3
  HH82/LConn1 -- Wire50/RConn1 -- Wire51/LConn1
  HH83/LConn1 -- Wire50/RConn2 -- Wire51/LConn2
  HH84/LConn1 -- Wire50/RConn3 -- Wire51/LConn3
  HH85/LConn1 -- Wire51/RConn1 -- Wire52/LConn1
  HH85/LConn2 -- Wire51/RConn2 -- Wire52/LConn2
  HH85/LConn3 -- Wire51/RConn3 -- Wire52/LConn3
  HH86/LConn1 -- Wire52/RConn1 -- Wire53/LConn1
  HH87/LConn1 -- Wire52/RConn2 -- Wire53/LConn2
  HH88/LConn1 -- Wire52/RConn3 -- Wire53/LConn3
  Wire53/RConn1 -- HH89/LConn1
  Wire53/RConn2 -- HH90/LConn1
  Wire53/RConn3 -- HH91/LConn1
  HH92/LConn1 -- Wire22/RConn1 -- Wire44/LConn1
  HH92/LConn2 -- Wire22/RConn2 -- Wire44/LConn2
  HH92/LConn3 -- Wire22/RConn3 -- Wire44/LConn3
  HH93/LConn1 -- Wire44/RConn1 -- Wire45/LConn1
  HH94/LConn1 -- Wire44/RConn2 -- Wire45/LConn2
  HH95/LConn1 -- Wire44/RConn3 -- Wire45/LConn3
  HH96/LConn1 -- Wire45/RConn1 -- Wire46/LConn1
  HH97/LConn1 -- Wire45/RConn2 -- Wire46/LConn2
  HH98/LConn1 -- Wire45/RConn3 -- Wire46/LConn3
  HH99/LConn1 -- Wire46/RConn1 -- Wire47/LConn1
  HH99/LConn2 -- Wire46/RConn2 -- Wire47/LConn2
  HH99/LConn3 -- Wire46/RConn3 -- Wire47/LConn3
  HH100/LConn1 -- Wire47/RConn1 -- Wire48/LConn1
  HH101/LConn1 -- Wire47/RConn2 -- Wire48/LConn2
  HH102/LConn1 -- Wire47/RConn3 -- Wire48/LConn3
  Wire48/RConn1 -- HH103/LConn1
  Wire48/RConn2 -- HH104/LConn1
  Wire48/RConn3 -- HH105/LConn1
  HH106/LConn1 -- Wire14/RConn1 -- Wire39/LConn1
  HH106/LConn2 -- Wire14/RConn2 -- Wire39/LConn2
  HH106/LConn3 -- Wire14/RConn3 -- Wire39/LConn3
  HH107/LConn1 -- Wire39/RConn1 -- Wire40/LConn1
  HH108/LConn1 -- Wire39/RConn2 -- Wire40/LConn2
  HH109/LConn1 -- Wire39/RConn3 -- Wire40/LConn3
  HH110/LConn1 -- Wire40/RConn1 -- Wire41/LConn1
  HH111/LConn1 -- Wire40/RConn2 -- Wire41/LConn2
  HH112/LConn1 -- Wire40/RConn3 -- Wire41/LConn3
  HH113/LConn1 -- Wire41/RConn1 -- Wire42/LConn1
  HH113/LConn2 -- Wire41/RConn2 -- Wire42/LConn2
  HH113/LConn3 -- Wire41/RConn3 -- Wire42/LConn3
  HH114/LConn1 -- Wire42/RConn1 -- Wire43/LConn1
  HH115/LConn1 -- Wire42/RConn2 -- Wire43/LConn2
  HH116/LConn1 -- Wire42/RConn3 -- Wire43/LConn3
  Wire43/RConn1 -- HH117/LConn1
  Wire43/RConn2 -- HH118/LConn1
  Wire43/RConn3 -- HH119/LConn1
  HH120/LConn1 -- Wire2/RConn1 -- Wire54/LConn1
  HH120/LConn2 -- Wire2/RConn2 -- Wire54/LConn2
  HH120/LConn3 -- Wire2/RConn3 -- Wire54/LConn3
  HH121/LConn1 -- Wire54/RConn1 -- Wire55/LConn1
  HH122/LConn1 -- Wire54/RConn2 -- Wire55/LConn2
  HH123/LConn1 -- Wire54/RConn3 -- Wire55/LConn3
  HH124/LConn1 -- Wire55/RConn1 -- Wire56/LConn1
  HH125/LConn1 -- Wire55/RConn2 -- Wire56/LConn2
  HH126/LConn1 -- Wire55/RConn3 -- Wire56/LConn3
  HH127/LConn1 -- Wire56/RConn1 -- Wire57/LConn1
  HH127/LConn2 -- Wire56/RConn2 -- Wire57/LConn2
  HH127/LConn3 -- Wire56/RConn3 -- Wire57/LConn3
  HH128/LConn1 -- Wire57/RConn1 -- Wire58/LConn1
  HH129/LConn1 -- Wire57/RConn2 -- Wire58/LConn2
  HH130/LConn1 -- Wire57/RConn3 -- Wire58/LConn3
  HH131/LConn1 -- Wire58/RConn1 -- Wire59/LConn1
  HH132/LConn1 -- Wire58/RConn2 -- Wire59/LConn2
  HH133/LConn1 -- Wire58/RConn3 -- Wire59/LConn3
  HH134/LConn1 -- Wire59/RConn1 -- Wire60/LConn1
  HH134/LConn2 -- Wire59/RConn2 -- Wire60/LConn2
  HH134/LConn3 -- Wire59/RConn3 -- Wire60/LConn3
  HH135/LConn1 -- Wire60/RConn1 -- Wire61/LConn1 -- Wire62/LConn1
  HH136/LConn1 -- Wire60/RConn2 -- Wire61/LConn2 -- Wire62/LConn2
  HH137/LConn1 -- Wire60/RConn3 -- Wire61/LConn3 -- Wire62/LConn3
  HH138/LConn1 -- Wire61/RConn1 -- Wire63/LConn1
  HH139/LConn1 -- Wire61/RConn2 -- Wire63/LConn2
  HH140/LConn1 -- Wire61/RConn3 -- Wire63/LConn3
  HH141/LConn1 -- Wire63/RConn1 -- Wire64/LConn1
  HH141/LConn2 -- Wire63/RConn2 -- Wire64/LConn2
  HH141/LConn3 -- Wire63/RConn3 -- Wire64/LConn3
  HH142/LConn1 -- Wire64/RConn1 -- Wire65/LConn1
  HH143/LConn1 -- Wire64/RConn2 -- Wire65/LConn2
  HH144/LConn1 -- Wire64/RConn3 -- Wire65/LConn3
  HH145/LConn1 -- Wire65/RConn1 -- Wire66/LConn1
  HH146/LConn1 -- Wire65/RConn2 -- Wire66/LConn2
  HH147/LConn1 -- Wire65/RConn3 -- Wire66/LConn3
  HH148/LConn1 -- Wire66/RConn1 -- Wire67/LConn1
  HH148/LConn2 -- Wire66/RConn2 -- Wire67/LConn2
  HH148/LConn3 -- Wire66/RConn3 -- Wire67/LConn3
  HH149/LConn1 -- Wire67/RConn1 -- Wire68/LConn1
  HH150/LConn1 -- Wire67/RConn2 -- Wire68/LConn2
  HH151/LConn1 -- Wire67/RConn3 -- Wire68/LConn3
  Wire68/RConn1 -- HH152/LConn1
  Wire68/RConn2 -- HH153/LConn1
  Wire68/RConn3 -- HH154/LConn1
  HH155/LConn1 -- Wire62/RConn1 -- Wire69/LConn1
  HH155/LConn2 -- Wire62/RConn2 -- Wire69/LConn2
  HH155/LConn3 -- Wire62/RConn3 -- Wire69/LConn3
  HH156/LConn1 -- Wire69/RConn1 -- Wire70/LConn1
  HH157/LConn1 -- Wire69/RConn2 -- Wire70/LConn2
  HH158/LConn1 -- Wire69/RConn3 -- Wire70/LConn3
  HH159/LConn1 -- Wire70/RConn1 -- Wire71/LConn1
  HH160/LConn1 -- Wire70/RConn2 -- Wire71/LConn2
  HH161/LConn1 -- Wire70/RConn3 -- Wire71/LConn3
  HH162/LConn1 -- Wire71/RConn1 -- Wire72/LConn1
  HH162/LConn2 -- Wire71/RConn2 -- Wire72/LConn2
  HH162/LConn3 -- Wire71/RConn3 -- Wire72/LConn3
  HH163/LConn1 -- Wire72/RConn1 -- Wire73/LConn1
  HH164/LConn1 -- Wire72/RConn2 -- Wire73/LConn2
  HH165/LConn1 -- Wire72/RConn3 -- Wire73/LConn3
  HH166/LConn1 -- Wire73/RConn1 -- Wire74/LConn1
  HH167/LConn1 -- Wire73/RConn2 -- Wire74/LConn2
  HH168/LConn1 -- Wire73/RConn3 -- Wire74/LConn3
  Wire74/RConn1 -- HH169/LConn1
  Wire74/RConn2 -- HH169/LConn2
  Wire74/RConn3 -- HH169/LConn3
  HH170/LConn1 -- Wire3/RConn1 -- Wire75/LConn1
  HH171/LConn1 -- Wire3/RConn2 -- Wire75/LConn2
  HH172/LConn1 -- Wire3/RConn3 -- Wire75/LConn3
  HH173/LConn1 -- Wire75/RConn1 -- Wire76/LConn1
  HH174/LConn1 -- Wire75/RConn2 -- Wire76/LConn2
  HH175/LConn1 -- Wire75/RConn3 -- Wire76/LConn3
  HH176/LConn1 -- Wire76/RConn1 -- Wire77/LConn1
  HH176/LConn2 -- Wire76/RConn2 -- Wire77/LConn2
  HH176/LConn3 -- Wire76/RConn3 -- Wire77/LConn3
  HH177/LConn1 -- Wire77/RConn1 -- Wire78/LConn1
  HH178/LConn1 -- Wire77/RConn2 -- Wire78/LConn2
  HH179/LConn1 -- Wire77/RConn3 -- Wire78/LConn3
  HH180/LConn1 -- Wire78/RConn1 -- Wire79/LConn1
  HH181/LConn1 -- Wire78/RConn2 -- Wire79/LConn2
  HH182/LConn1 -- Wire78/RConn3 -- Wire79/LConn3
  HH183/LConn1 -- Wire79/RConn1 -- Wire80/LConn1
  HH183/LConn2 -- Wire79/RConn2 -- Wire80/LConn2
  HH183/LConn3 -- Wire79/RConn3 -- Wire80/LConn3
  HH184/LConn1 -- Wire80/RConn1 -- Wire81/LConn1
  HH185/LConn1 -- Wire80/RConn2 -- Wire81/LConn2
  HH186/LConn1 -- Wire80/RConn3 -- Wire81/LConn3
  HH187/LConn1 -- Wire81/RConn1 -- Wire82/LConn1
  HH188/LConn1 -- Wire81/RConn2 -- Wire82/LConn2
  HH189/LConn1 -- Wire81/RConn3 -- Wire82/LConn3
  HH190/LConn1 -- Wire82/RConn1 -- Wire83/LConn1
  HH190/LConn2 -- Wire82/RConn2 -- Wire83/LConn2
  HH190/LConn3 -- Wire82/RConn3 -- Wire83/LConn3
  HH191/LConn1 -- Wire83/RConn1 -- Wire84/LConn1
  HH192/LConn1 -- Wire83/RConn2 -- Wire84/LConn2
  HH193/LConn1 -- Wire83/RConn3 -- Wire84/LConn3
  HH194/LConn1 -- Wire84/RConn1 -- Wire85/LConn1
  HH195/LConn1 -- Wire84/RConn2 -- Wire85/LConn2
  HH196/LConn1 -- Wire84/RConn3 -- Wire85/LConn3
  HH197/LConn1 -- Wire85/RConn1 -- Wire86/LConn1
  HH197/LConn2 -- Wire85/RConn2 -- Wire86/LConn2
  HH197/LConn3 -- Wire85/RConn3 -- Wire86/LConn3
  HH198/LConn1 -- Wire86/RConn1 -- Wire87/LConn1
  HH199/LConn1 -- Wire86/RConn2 -- Wire87/LConn2
  HH200/LConn1 -- Wire86/RConn3 -- Wire87/LConn3
  Wire87/RConn1 -- Wire88/LConn1
  Wire87/RConn2 -- Wire88/LConn2
  Wire87/RConn3 -- Wire88/LConn3
  Wire88/RConn1 -- HH201/LConn1
  Wire88/RConn2 -- HH201/LConn2
  Wire88/RConn3 -- HH201/LConn3
